simulink model "fftanalyzeri"  (R2012b)
settings: Solver=ode3  SolverMode=SingleTasking  StartTime=0.0  StopTime=20000  RelTol=1e-3
undefined symbols (not defined in the file or in its folder): pfb_coeff_gen_calc
undefined symbols (not defined in the file): fft_bin_flags_, magphmeanmem_, threshmem_
libraries: xbsIndex_r4 x9073, casper_library_misc x119, casper_library_flow_control x51, casper_library_delays x22, xps_library x10
(part 1 of 74)
settings Model: Creator=tmadden  LastModifiedBy=tmadden

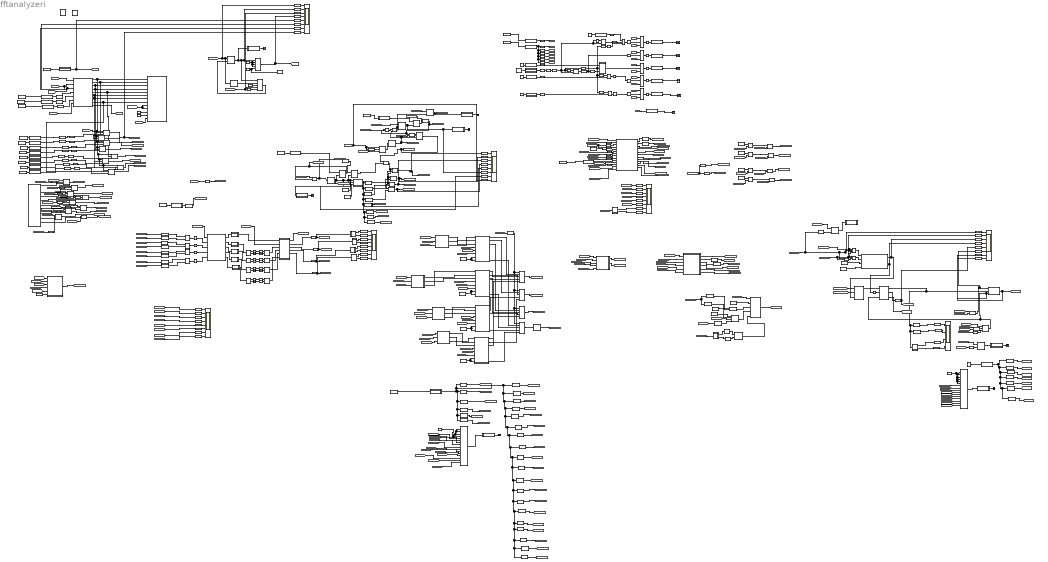
== system fftanalyzeri ==
  note: dumopFIFO is reallty read out fifos in proper wa to store fft data
  note: means fftcnt NOT done
  note: 32bits
  note: 32bits
  note: 32bits
  note: 32bits
  note: 7bits
  note: 0x55
  note: 16bits
  note: 16bits
  note: 16 bits
  note: 1bit
  note: 8 buts
  note: 0xaaaa
  note: 1st word fall thru
  note: 32 bit timestamp
  note: Now we put data backtogether
      | into 32bit buss
  note: This block extracts mag and phase
      | but truncates both numbers
      | to 16 bit.
  note: WE shrunk the mem to total of 32 bits
      | so we dont use all the bits in
      | header info.
      | all coef data go thru, but gets
      | truncated later...
      | we shoudl truncate here
      | to save resources...
  note: We truncate to 16bit data.
      | power is unsigned, all fraction bits
      | phase is signed w/ 13 frac bits
  note: This reg and bits are for
      | python user interface control
  note: if dropall evetns is 1 then save event and delete event will cause
      | a event to be deleted.
      | if drop all evetns is 0 then save event saves and delete events
      | deletes
  note: Because of bug in the fifos
      | we need extra delay on dvld.
      | we should out then in all
      | the underlying f16 chan fifos.
      | This is simpler for now...
  note: 1024 long
      | 32 bit wide
  note: 2 bits, sel 0,1,2,3 fifo
  note: Alolow fake ADC data to come into the system
  note: Counts number of FFTs forever
  note: if we want neg freq, that is freq below the rf carrier
      | we piuck eith coef 128-255 or 384 to 511
  note: ecause we cant read in whole fft we sel neg or pos freq
      | therefore we have a mux to give us coef 0-127 OR 256-383
  note: when startFFTs go high, cnt goes to state 0
      | when startFFt go low, cnt will goto state 1 because
      | of delayed 1 in delay19. counter gets to 2
      | and waits for lutsync, then goto 3.
      | it staty in 3 until we startFFTs again.
      | to shut ffts, set startFFTs high forever.
  note: Or a simulation input w/ HW input. the LIT is wierd in sumulation...
  note: go high to turn ffts mem storage off.
      | Go low to sync fft sunc to lut for phse reference
      | start fft saving
  note: states
      | 0	wait for fftstmem to go low, no fft sync
      | 1 waut for fftmemwe 0->1, no fft sunc
      | 2 wait for lut sync, no fft sunc
      | 3 fft sunc on, stay in this state forever
      |
      | fftstmem, forces fsm to state 0
  note: syscunc=1
      | startdac=0
      | startdac=1
      | syscunc=0
  note: if run_ffts is high, then the ffts run. else no ffts run.
  note: Read out FIFO state machine. Sauy we have 128 bins from fft. We read in groups of 4, w/ 4 outputs, so each fifo gets 32 bins
      | in each. So we will read out 32 numbers from each fifo. Counter counts from 0 to 127. LSBs pick which fifo.
      | There is a pipe line here. 1st we trigger FFT, which writes to FIFOS. Also we truggerm, assuming 1 fft pipeline delay
      | radoung out fifos. We have to read and write fifos same number of times or else we get out of sync
  note: The above is Ran's design for  ROACH IF baord
      | serial data stream. For programming IF board
      | clocks, gains, dividers.
  note: SWAT_LE
  note: LO_SLE
  note: SER_DI
  note: SER_CLK
  note: SW_STB
  note: Added by Tim Madden
  note: not in RANS design- below. Tim added the clk sle register so we can program the clocks
  note: bit 7
  note: CLK_SLE
  note: If bin>512, we disable any write fifo bits.
      | high if IS VALID bin number
  note: address for multi-fifo- which fifo does thei bin go into.
  note: Hight if we have computed less then N ffts
  note: just started daq, reset fft cnt to 0
  note: increments fft counter
  note: pulse for 1st fft done after starting daq
  note: pulse for every fft
  note: When high, we can write fifos, and read fifos, and wr end mdmory
  note: We can compute N ffts and stop storong.
      | This counts ffts stored.
      | Counter is reset on runffts going high,.
      | it is incremented every time we compute a fft.
  note: Set of 1's and 0;s in lsb
      | 1 to write that fft coef to fifos.
      | 4 outputs for fft, so we ave 4 bits
      | to det. if we write coef to fifo
  note: Bin counter.
      | inc for ecah bin from 0 to 511, or
      | mult of 512-1 up to 4k.when count
      | to 511, we write EVERY fft.
      | if we count to 1023, we write every other fft,
      | as long as the mem in BinData is 0 uip there.
      | We assume it is.
  note: high for each coef to write to fifo
  note: This is a pulse of 1 clk, for every group of coeffs to write. one pulse per ffft. goes 1 , 1clk before 1st coef
  note: This tunrs on after fftcuncout and staus on. as long as runffts is high.
  note: This Must be multiple of 512-1, like 511,1023,2047, max is 32 bits...
      | It can then skip FFTS, as higher mem on BinData is set to 0.
      | In thys way the 512 coef from FFT get written every Nth time. This is good if we wish to slow sample rate, or read whol FFT
      | Set to 512*5 - 1 to safely read all FFT coef.
  note: run_ffts is low, then q is 0.
      | run_ffts is hi, then q is one after fftsuncout.
      | this allows fifl wr
      | We can only write fifos when run_ffts is high.
      | fftoutsync comes some time after run-ffts goes high, when fft is done
  note: This is bin counter. it resets to 0 after 511, so it goes 0,1,2,3...511,0,1,2
      | it resets on fftsunc out, which happens once on reset at start of collection
  note: fftsyncout comes once at start of collection.
      | 1 clk lengthn pulse
      | it is for resetting and starting data collection
  note: Line up w/ data.
      | t1, fftdata0
      | tt4, phase 0
  note: fftsyncout_____________--________
  note: t=0,0
      | t=1,0
      | t=2,1
      | t=258,0
  note: at t=0, rst=1
      | t=1, cnt=0
      | t=2 cnt=1
      | t=257,cnt=256,
      | t=258...cnt=256
  note: FFT tap0: fft bin   04,8,etc.
      | tap 1  1,5,9...
      | tap 2   2,6,10...
      | tap3   3,7,11
  note: does mnothing.. set to 0
  note: run script fft_simvals.m to get this var
  note: 1 to let dac work
  note: make lut output the dram address instead if contents
  note: 1 to allow writing fft coef to fifos and output mem
  note: reset lut i think
  note: reset fft coef output mem addr to zero
  note: force fifo read to empty fifo of bad data
  note: loops back lut data into ffts, bypassing dac/adc etc
  note: set to 1 to make things run
  note: set whehc data gets saved to adc mem
  note: enable saving adc data to mem
  note: set adc wavemem addr to 0
  note: 1,0 will sync ffts w/ LUT and enable saving fft coef to ram
  note: Delay data, so we can save data befpre pulse was triggered
  note: Delay the data balid signal and data, so the pulse detector leads te actual data.
      | in this way we can detect pulse, shut off fifo, write header, then write the
      | 1st sample taht triggered pulse to memory
  note: Insert header data before pulse data.
      | We write just pulses to outptu memory.
      | So before pulse, we write magix number of 64k,
      | then write channel number,
      | then output pulse data.
  note: 32kx16bit
  note: 32K outptu fifo
      | uses ded. fifo
      | 32kwords * 4.5bytes/word=144kB
      | 16k length---> 72kB
  note: We read big fifo, and write to outram on this condition:
      | out ram is not full
      | we have NON empty fifo, that is, data is available from big fifo
      | We have enabled outmem writing w/ fftMemWE=1
  note: 1 when mem is full.
  note: fftMemWE enables reading 32K fifo into outram.
      | if memdone is high, we will not read the 32k fifo.
      | We read the big filo by
      | 1. fftMemWE<=0
      | 2. stFFTMem<=1
      | 3. stFFTMem<=0
      | 4 fftMemWE<=1
      | The fifo will be read, as long as there is data in it, until the outmem fills
      | or we set fftMemWE to 0.
      | When MemDone is 1, then we set fftMemWE to 0
      | We then copy memory w./ python over the network to linux.
      | Then we got to steo 1.
  note: 32k x 16bit
  note: Reset output mem addr to 0.
  note: wrout
  note: empty
  note: Output mempry that stores headers/pulse data.
      | Events to be written back to linux box.
  " System Generator" : xbsIndex_r4/ System Generator  Tag=genX  xilinxfamily=virtex5  part=xc5vsx95t  speed=-1  package=ff1136  synthesis_tool=XST  clock_wrapper=Clock Enables  directory=./fftanalyzeri/sysgen  proj_type=Project Navigator  Synth_file=XST Defaults  Impl_file=ISE Defaults  testbench=off  simulink_period=1  sysclk_period=7.8125  dcm_input_clock_period=100  incr_netlist=off  trim_vbits=Everywhere in SubSystem  dbl_ovrd=According to Block Masks  core_generation=According to Block Masks  run_coregen=off  deprecated_control=off  eval_field=0  block_type=sysgen
  Assert{,1..3} (4 alike) : xbsIndex_r4/Assert  assert_type=on  type_source=Explicitly  gui_display_data_type=Boolean  arith_type=Boolean  n_bits=16  bin_pt=14  preci_type=Single  exp_width=8  frac_width=24  assert_rate=on  rate_source=Explicitly  period=1  output_port=on  block_type=assert
  BinCounter : xbsIndex_r4/Counter  cnt_type=Free Running  cnt_to=Inf  operation=Up  start_count=0  cnt_by_val=1  arith_type=Unsigned  n_bits=32  bin_pt=0  load_pin=off  rst=on  en=off  explicit_period=on  period=1  dbl_ovrd=off  use_behavioral_HDL=off  implementation=Fabric  block_type=counter
  BinData : Subsystem  Tag=xps:bram  AncestorBlock=xps_library/Shared BRAM  mask{arith_type=Unsigned, addr_width=10, data_width=32, reg_prim_output=off, reg_core_output=off, optimization=Minimum_Area, data_bin_pt=0, init_vals=fft_bin_flags_, sample_rate=1}
      mask prompts: arith_type "Output Data Type"; addr_width "Address width"; data_width "Data Width"; reg_prim_output "Register Primitive Output"; reg_core_output "Register Core Output"; data_bin_pt "Data Binary Point"; init_vals "Initial values (simulation only)"; sample_rate "Sample rate"
      mask init:
      | shared_bram_mask;
      mask TypeOptions arith_type: Unsigned | Signed  (2's comp)
      mask TypeOptions data_width: 8 | 16 | 32 | 64 | 128
      mask TypeOptions optimization: Minimum_Area | Low_Power
  Concat : xbsIndex_r4/Concat  num_inputs=16  dbl_ovrd=off  block_type=concat
  Concat1 : xbsIndex_r4/Concat  num_inputs=4  dbl_ovrd=off  block_type=concat
  Concat2 : xbsIndex_r4/Concat  num_inputs=2  dbl_ovrd=off  block_type=concat
  Concat3 : xbsIndex_r4/Concat  num_inputs=16  dbl_ovrd=off  block_type=concat
  Concat4 : xbsIndex_r4/Concat  num_inputs=2  dbl_ovrd=off  block_type=concat
  Constant : xbsIndex_r4/Constant  const=0  gui_display_data_type=Boolean  arith_type=Boolean  n_bits=16  bin_pt=14  preci_type=Single  exp_width=8  frac_width=24  explicit_period=on  period=1  equ=P=C  opselect=C  inp2=PCIN>>17  opr=+  inp1=P  carry=CIN  dbl_ovrd=off  block_type=constant
  Constant1 : xbsIndex_r4/Constant  const=0  gui_display_data_type=Fixed-point  arith_type=Unsigned  n_bits=8  bin_pt=0  preci_type=Single  exp_width=8  frac_width=24  explicit_period=on  period=1  equ=P=C  opselect=C  inp2=PCIN>>17  opr=+  inp1=P  carry=CIN  dbl_ovrd=off  block_type=constant
  Constant10 : xbsIndex_r4/Constant  const=0  gui_display_data_type=Boolean  arith_type=Boolean  n_bits=4  bin_pt=0  preci_type=Single  exp_width=8  frac_width=24  explicit_period=on  period=1  equ=P=C  opselect=C  inp2=PCIN>>17  opr=+  inp1=P  carry=CIN  dbl_ovrd=off  block_type=constant
      settings: block_version=11.4
  Constant11 : Constant
  Constant12 : Constant  Value=2^31 + 2^29 + 2^15+2^4 + 2^0
  Constant14 : Constant
  Constant15 : Constant
  Constant2 : xbsIndex_r4/Constant  const=0  gui_display_data_type=Boolean  arith_type=Boolean  n_bits=4  bin_pt=0  preci_type=Single  exp_width=8  frac_width=24  explicit_period=on  period=1  equ=P=C  opselect=C  inp2=PCIN>>17  opr=+  inp1=P  carry=CIN  dbl_ovrd=off  block_type=constant
      settings: block_version=11.4
  Constant20 : xbsIndex_r4/Constant  const=0  gui_display_data_type=Boolean  arith_type=Boolean  n_bits=8  bin_pt=0  preci_type=Single  exp_width=8  frac_width=24  explicit_period=on  period=1  equ=P=C  opselect=C  inp2=PCIN>>17  opr=+  inp1=P  carry=CIN  dbl_ovrd=off  block_type=constant
  Constant24 : xbsIndex_r4/Constant  const=0  gui_display_data_type=Fixed-point  arith_type=Boolean  n_bits=4  bin_pt=0  preci_type=Single  exp_width=8  frac_width=24  explicit_period=on  period=1  equ=P=C  opselect=C  inp2=PCIN>>17  opr=+  inp1=P  carry=CIN  dbl_ovrd=off  block_type=constant
      settings: block_version=11.4
  Constant25 : xbsIndex_r4/Constant  const=1  gui_display_data_type=Boolean  arith_type=Boolean  n_bits=4  bin_pt=0  preci_type=Single  exp_width=8  frac_width=24  explicit_period=on  period=1  equ=P=C  opselect=C  inp2=PCIN>>17  opr=+  inp1=P  carry=CIN  dbl_ovrd=off  block_type=constant
      settings: block_version=11.4
  Constant26 : xbsIndex_r4/Constant  const=1  gui_display_data_type=Boolean  arith_type=Boolean  n_bits=4  bin_pt=0  preci_type=Single  exp_width=8  frac_width=24  explicit_period=on  period=1  equ=P=C  opselect=C  inp2=PCIN>>17  opr=+  inp1=P  carry=CIN  dbl_ovrd=off  block_type=constant
      settings: block_version=11.4
  Constant3 : Constant  Value=0
  Constant6 : xbsIndex_r4/Constant  const=0  gui_display_data_type=Fixed-point  arith_type=Boolean  n_bits=4  bin_pt=0  preci_type=Single  exp_width=8  frac_width=24  explicit_period=on  period=1  equ=P=C  opselect=C  inp2=PCIN>>17  opr=+  inp1=P  carry=CIN  dbl_ovrd=off  block_type=constant
      settings: block_version=11.4
  Constant7 : xbsIndex_r4/Constant  const=0  gui_display_data_type=Fixed-point  arith_type=Boolean  n_bits=4  bin_pt=0  preci_type=Single  exp_width=8  frac_width=24  explicit_period=on  period=1  equ=P=C  opselect=C  inp2=PCIN>>17  opr=+  inp1=P  carry=CIN  dbl_ovrd=off  block_type=constant
      settings: block_version=11.4
  Constant8 : xbsIndex_r4/Constant  const=0  gui_display_data_type=Fixed-point  arith_type=Unsigned  n_bits=4  bin_pt=0  preci_type=Single  exp_width=8  frac_width=24  explicit_period=on  period=1  equ=P=C  opselect=C  inp2=PCIN>>17  opr=+  inp1=P  carry=CIN  dbl_ovrd=off  block_type=constant
      settings: block_version=11.4
  Convert{4,6..12} (8 alike) : xbsIndex_r4/Convert  gui_display_data_type=Fixed-point  arith_type="Signed  (2's comp)"  n_bits=18  bin_pt=17  float_type=Single  exp_bits=8  fraction_bits=24  quantization="Round  (unbiased: +/- Inf)"  overflow=Wrap  en=off  latency=0  dbl_ovrd=off  pipeline=off  block_type=convert
      settings: xl_area=[0 0 0 0 0 0 0]  block_version=10.1.3
  Convert5 : xbsIndex_r4/Convert  gui_display_data_type=Fixed-point  arith_type=Unsigned  n_bits=33  bin_pt=0  float_type=Single  exp_bits=8  fraction_bits=24  quantization=Truncate  overflow=Wrap  en=off  latency=0  dbl_ovrd=off  pipeline=off  block_type=convert
      settings: block_version=11.4
  Counter2 : xbsIndex_r4/Counter  cnt_type=Free Running  cnt_to=2048  operation=Up  start_count=0  cnt_by_val=1  arith_type=Unsigned  n_bits=8  bin_pt=0  load_pin=off  rst=on  en=on  explicit_period=on  period=1  dbl_ovrd=off  use_behavioral_HDL=off  implementation=Fabric  use_rpm=off  block_type=counter
  Counter4 : xbsIndex_r4/Counter  cnt_type=Free Running  cnt_to=Inf  operation=Up  start_count=0  cnt_by_val=1  arith_type=Unsigned  n_bits=8  bin_pt=0  load_pin=off  rst=on  en=on  explicit_period=on  period=1  dbl_ovrd=off  use_behavioral_HDL=off  implementation=Fabric  block_type=counter
      settings: block_version=11.4
  DRAM_LUT : Subsystem
  DSbit0 : xbsIndex_r4/Slice  nbits=1  boolean_output=on  mode=Lower Bit Location + Width  bit1=0  base1=MSB of Input  bit0=0  base0=LSB of Input  dbl_ovrd=off  block_type=slice
  DSbit1 : xbsIndex_r4/Slice  nbits=1  boolean_output=on  mode=Lower Bit Location + Width  bit1=0  base1=MSB of Input  bit0=1  base0=LSB of Input  dbl_ovrd=off  block_type=slice
  DSbit2 : xbsIndex_r4/Slice  nbits=1  boolean_output=on  mode=Lower Bit Location + Width  bit1=0  base1=MSB of Input  bit0=2  base0=LSB of Input  dbl_ovrd=off  block_type=slice
  DSbit3 : xbsIndex_r4/Slice  nbits=1  boolean_output=on  mode=Lower Bit Location + Width  bit1=0  base1=MSB of Input  bit0=3  base0=LSB of Input  dbl_ovrd=off  block_type=slice
  DSbit4 : xbsIndex_r4/Slice  nbits=1  boolean_output=on  mode=Lower Bit Location + Width  bit1=0  base1=MSB of Input  bit0=4  base0=LSB of Input  dbl_ovrd=off  block_type=slice
  DSbit5 : xbsIndex_r4/Slice  nbits=1  boolean_output=on  mode=Lower Bit Location + Width  bit1=0  base1=MSB of Input  bit0=5  base0=LSB of Input  dbl_ovrd=off  block_type=slice
  DSbit6 : xbsIndex_r4/Slice  nbits=1  boolean_output=on  mode=Lower Bit Location + Width  bit1=0  base1=MSB of Input  bit0=6  base0=LSB of Input  dbl_ovrd=off  block_type=slice
  Delay{,2,9..16,18,20,29..32,34} (17 alike) : xbsIndex_r4/Delay  rst=off  infoeditControl=Selection of Reset will increase slice count due to use of real FFs and instead of SRLs  en=off  latency=1  dbl_ovrd=off  reg_retiming=off  block_type=delay
      Delay10 settings: xl_area=[18 36 0 0 0 0 0]
      Delay11 settings: xl_area=[18 36 0 0 0 0 0]
      Delay12 settings: xl_area=[18 36 0 0 0 0 0]
      Delay9 settings: xl_area=[18 36 0 0 0 0 0]
  Delay{1,3..8,17,19,21} (10 alike) : xbsIndex_r4/Delay  rst=off  infoeditControl=Selection of Reset will increase slice count due to use of real FFs and instead of SRLs  en=off  latency=2  dbl_ovrd=off  reg_retiming=off  block_type=delay
  Delay{23..24,27..28} (4 alike) : xbsIndex_r4/Delay  rst=off  infoeditControl=Selection of Reset will increase slice count due to use of real FFs and instead of SRLs  en=off  latency=64  dbl_ovrd=off  reg_retiming=off  block_type=delay
      settings: block_version=11.4
  EventLength : xbsIndex_r4/Constant  const=34  gui_display_data_type=Fixed-point  arith_type=Unsigned  n_bits=8  bin_pt=0  preci_type=Single  exp_width=8  frac_width=24  explicit_period=on  period=1  equ=P=C  opselect=C  inp2=PCIN>>17  opr=+  inp1=P  carry=CIN  dbl_ovrd=off  block_type=constant
  EventSaveFSM : xbsIndex_r4/MCode  mfname=eventsaveFSM  explicit_period=off  period=1  inputsTable={'boundInpExpr'=>['','','',''],'inputs'=>['save_event','delete_event','event_length','rst']}  outputsTable={'outputs'=>['eventfifo_rd','outfifo_wr'],'suppressOut'=>['off','off']}  dbl_ovrd=off  enable_stdout=off  enable_debug=off  suppress_output=on  defparams={}  hide_port_list={}  block_type=mcode
  EvtCnt : xbsIndex_r4/Counter  cnt_type=Free Running  cnt_to=Inf  operation=Up  start_count=0  cnt_by_val=1  arith_type=Unsigned  n_bits=32  bin_pt=0  load_pin=off  rst=on  en=on  explicit_period=on  period=1  dbl_ovrd=off  use_behavioral_HDL=off  implementation=Fabric  block_type=counter
  FIFO64_ : Subsystem
  FIFO64_1 : Subsystem
  FIFO64_2 : Subsystem
  FIFO64_3 : Subsystem
  From Workspace : FromWorkspace  VariableName=controlReg  OutDataTypeStr=double  SampleTime=1  Interpolate=off  OutputAfterFinalValue=Holding final value
  From Workspace1 : FromWorkspace  VariableName=if_switch  SampleTime=1  Interpolate=off  OutputAfterFinalValue=Holding final value
  From Workspace10 : FromWorkspace  VariableName=LUTsize  SampleTime=1  Interpolate=off  OutputAfterFinalValue=Holding final value
  From Workspace11 : FromWorkspace  VariableName=lut_i0  SampleTime=1  Interpolate=off  OutputAfterFinalValue=Holding final value
  From Workspace12 : FromWorkspace  VariableName=lut_i1  SampleTime=1  Interpolate=off  OutputAfterFinalValue=Holding final value
  From Workspace13 : FromWorkspace  VariableName=lut_i2  SampleTime=1  Interpolate=off  OutputAfterFinalValue=Holding final value
  From Workspace14 : FromWorkspace  VariableName=lut_i3  SampleTime=1  Interpolate=off  OutputAfterFinalValue=Holding final value
  From Workspace15 : FromWorkspace  VariableName=lut_q0  SampleTime=1  Interpolate=off  OutputAfterFinalValue=Holding final value
  From Workspace16 : FromWorkspace  VariableName=lut_q1  SampleTime=1  Interpolate=off  OutputAfterFinalValue=Holding final value
  From Workspace17 : FromWorkspace  VariableName=lut_q2  SampleTime=1  Interpolate=off  OutputAfterFinalValue=Holding final value
  From Workspace18 : FromWorkspace  VariableName=lut_q3  SampleTime=1  Interpolate=off  OutputAfterFinalValue=Holding final value
  From Workspace2 : FromWorkspace  VariableName=regs  SampleTime=1  Interpolate=off  OutputAfterFinalValue=Holding final value
  From Workspace3 : FromWorkspace  VariableName=lastChanToRead  SampleTime=1  Interpolate=off  OutputAfterFinalValue=Holding final value
  From Workspace4 : FromWorkspace  VariableName=numffts  SampleTime=1  Interpolate=off  OutputAfterFinalValue=Holding final value
  From Workspace5 : FromWorkspace  VariableName=fftsynctime  SampleTime=1  Interpolate=off  OutputAfterFinalValue=Holding final value
  From Workspace6 : FromWorkspace  VariableName=fftshift  SampleTime=1  Interpolate=off  OutputAfterFinalValue=Holding final value
  From Workspace7 : FromWorkspace  VariableName=resetDRAM  SampleTime=1  Interpolate=off  OutputAfterFinalValue=Holding final value
  From Workspace8 : FromWorkspace  VariableName=RWen  SampleTime=1  Interpolate=off  OutputAfterFinalValue=Holding final value
  From Workspace9 : FromWorkspace  VariableName=holdcounter  SampleTime=1  Interpolate=off  OutputAfterFinalValue=Holding final value
  Gateway Out{,1..51} (52 alike) : xbsIndex_r4/Gateway Out  inherit_from_input=off  hdl_port=on  timing_constraint=None  locs_specified=off  LOCs={}  UseAsDAC=off  DACChannel='1'  block_type=gatewayout
  Inverter{,1..6,8} (8 alike) : xbsIndex_r4/Inverter  en=off  latency=0  dbl_ovrd=off  block_type=inv
      Inverter1 settings: block_version=11.4
      Inverter2 settings: block_version=11.4
      Inverter3 settings: block_version=11.4
      Inverter4 settings: block_version=11.4
      Inverter5 settings: block_version=11.4
  LO_SLE : Subsystem  Tag=xps:sw_reg  AncestorBlock=xps_library/software register  mask{numios=1, io_dir=From Processor, io_delay=0, sample_period=1, name1=reg, bitwidth1=32, arith_type1=Unsigned, bin_pt1=0}
      mask prompts: numios "Num I/Os"; io_dir "I/O direction"; io_delay "I/O delay"; sample_period "Sample period"; name1 "Name"; bitwidth1 "Bitwidth"; arith_type1 "Type"; bin_pt1 "Binary pt"
      mask init:
      | swreg_init(gcb);
      mask Callback numios: t = timer('StartDelay', 0.1); t.TimerFcn = {@swreg_cb, gcb}; start(t);
      mask TypeOptions io_dir: To Processor | From Processor
      mask Callback io_dir:
      | a = get_param(gcb, 'MaskEnables');
      | if strcmp(get_param(gcb, 'io_dir'), 'To Processor'),
      | a(4) = {'off'};
      | else
      | a(4) = {'on'};
      | end
      | set_param(gcb, 'MaskEnables', a);
      mask TypeOptions arith_type1: Unsigned | Signed  (2's comp) | Boolean
      mask Callback arith_type1:
      | a = get_param(gcb, 'MaskEnables');
      | if strcmp(get_param(gcb, 'arith_type1'), 'Boolean'),
      | set_param(gcb, 'bitwidth1', '1');
      | set_param(gcb, 'bin_pt1', '0');
      | a(6) = {'off'};
      | a(8) = {'off'};
      | else
      | a(6) = {'on'};
      | a(8) = {'on'};
      | end
      | set_param(gcb, 'MaskEnables', a);
  LUTsize : Subsystem  Tag=xps:sw_reg  AncestorBlock=xps_library/software register  mask{numios=1, io_dir=From Processor, io_delay=0, sample_period=1, name1=reg, bitwidth1=32, arith_type1=Unsigned, bin_pt1=0}
      mask prompts: numios "Num I/Os"; io_dir "I/O direction"; io_delay "I/O delay"; sample_period "Sample period"; name1 "Name"; bitwidth1 "Bitwidth"; arith_type1 "Type"; bin_pt1 "Binary pt"
      mask init:
      | swreg_init(gcb);
      mask Callback numios: t = timer('StartDelay', 0.1); t.TimerFcn = {@swreg_cb, gcb}; start(t);
      mask TypeOptions io_dir: To Processor | From Processor
      mask Callback io_dir:
      | a = get_param(gcb, 'MaskEnables');
      | if strcmp(get_param(gcb, 'io_dir'), 'To Processor'),
      | a(4) = {'off'};
      | else
      | a(4) = {'on'};
      | end
      | set_param(gcb, 'MaskEnables', a);
      mask TypeOptions arith_type1: Unsigned | Signed  (2's comp) | Boolean
      mask Callback arith_type1:
      | a = get_param(gcb, 'MaskEnables');
      | if strcmp(get_param(gcb, 'arith_type1'), 'Boolean'),
      | set_param(gcb, 'bitwidth1', '1');
      | set_param(gcb, 'bin_pt1', '0');
      | a(6) = {'off'};
      | a(8) = {'off'};
      | else
      | a(6) = {'on'};
      | a(8) = {'on'};
      | end
      | set_param(gcb, 'MaskEnables', a);
  Logical : xbsIndex_r4/Logical  logical_function=AND  inputs=3  en=off  latency=0  precision=Full  arith_type=Unsigned  n_bits=16  bin_pt=0  align_bp=on  dbl_ovrd=off  block_type=logical
  Logical{1..3,14..17} (7 alike) : xbsIndex_r4/Logical  logical_function=OR  inputs=2  en=off  latency=0  precision=Full  arith_type=Unsigned  n_bits=16  bin_pt=0  align_bp=on  dbl_ovrd=off  block_type=logical
  Logical{4..8,10..13} (9 alike) : xbsIndex_r4/Logical  logical_function=AND  inputs=2  en=off  latency=0  precision=Full  arith_type=Unsigned  n_bits=16  bin_pt=0  align_bp=on  dbl_ovrd=off  block_type=logical
      Logical7 settings: block_version=11.4
      Logical8 settings: block_version=11.4
  Logical9 : xbsIndex_r4/Logical  logical_function=AND  inputs=3  en=off  latency=0  precision=Full  arith_type=Unsigned  n_bits=16  bin_pt=0  align_bp=on  dbl_ovrd=off  block_type=logical
      settings: block_version=11.4
  MCode1 : xbsIndex_r4/MCode  mfname=fifoFSMPh  explicit_period=on  period=1  inputsTable={'boundInpExpr'=>['','','','','','','','','','','','',''],'inputs'=>['dumpFifo','fifo_empty','half_full','quart_full','almost_full','rst','proc_busy','is_pulse','data_valid','last_channel','wr_raw_data','ram_pulse_state','is_calc_mean']}  outputsTable={'outputs'=>['fifo_rden','wr_coef_big_fifo','write_data_sel','cur_chanout','fifo_overrun_cnt_out','stateout','clear_pulse','datapath_enable','save_event','delete_event','save_pulse_state','calc_mean','store_mean'],'suppressOut'=>['off','off','off','off','off','off','off','off','off','off','off','off','off']}  dbl_ovrd=off  enable_stdout=off  enable_debug=off  suppress_output=on  defparams={}  hide_port_list={}  block_type=mcode
  MemRecordPolar : Subsystem
  Mux{,1..20} (21 alike) : xbsIndex_r4/Mux  inputs=2  en=off  latency=1  precision=Full  arith_type=Unsigned  n_bits=16  bin_pt=14  quantization=Truncate  overflow=Wrap  dbl_ovrd=off  block_type=mux
      Mux2 settings: block_version=11.4
      Mux3 settings: block_version=11.4
      Mux4 settings: block_version=11.4
      Mux5 settings: block_version=11.4
      Mux6 settings: block_version=11.4
  Mux21 : xbsIndex_r4/Mux  inputs=4  en=off  latency=0  precision=Full  arith_type=Unsigned  n_bits=16  bin_pt=14  quantization=Truncate  overflow=Wrap  dbl_ovrd=off  block_type=mux
  Mux22 : xbsIndex_r4/Mux  inputs=2  en=off  latency=0  precision=Full  arith_type=Unsigned  n_bits=16  bin_pt=14  quantization=Truncate  overflow=Wrap  dbl_ovrd=off  block_type=mux
  Mux23 : xbsIndex_r4/Mux  inputs=2  en=off  latency=0  precision=Full  arith_type=Unsigned  n_bits=16  bin_pt=14  quantization=Truncate  overflow=Wrap  dbl_ovrd=off  block_type=mux
  OutFIFO : xbsIndex_r4/FIFO  mem_type=Built-in FIFO  performance_options=First_Word_Fall_Through  infoedit1=Available only for V4, V5, V6, V7, K7, A7 and Zynq devices.  embedded_registers=off  depth=32K  percent_nbits=1  rst=off  en=off  use_dcount=off  use_percent_full_port=off  use_almost_empty=off  almost_empty_thresh=2  use_almost_full=off  almost_full_thresh=14  dbl_ovrd=off  explicit_period=off  block_type=fifo
  PhaseCorrect1 : Subsystem
  Pulse Generator2 : DiscretePulseGenerator  Period=11000  PulseWidth=10000  PhaseDelay=100
  PulseDetector : Subsystem
  RWen : Subsystem  Tag=xps:sw_reg  AncestorBlock=xps_library/software register  mask{numios=1, io_dir=From Processor, io_delay=0, sample_period=1, name1=reg, bitwidth1=32, arith_type1=Unsigned, bin_pt1=0}
      mask prompts: numios "Num I/Os"; io_dir "I/O direction"; io_delay "I/O delay"; sample_period "Sample period"; name1 "Name"; bitwidth1 "Bitwidth"; arith_type1 "Type"; bin_pt1 "Binary pt"
      mask init:
      | swreg_init(gcb);
      mask Callback numios: t = timer('StartDelay', 0.1); t.TimerFcn = {@swreg_cb, gcb}; start(t);
      mask TypeOptions io_dir: To Processor | From Processor
      mask Callback io_dir:
      | a = get_param(gcb, 'MaskEnables');
      | if strcmp(get_param(gcb, 'io_dir'), 'To Processor'),
      | a(4) = {'off'};
      | else
      | a(4) = {'on'};
      | end
      | set_param(gcb, 'MaskEnables', a);
      mask TypeOptions arith_type1: Unsigned | Signed  (2's comp) | Boolean
      mask Callback arith_type1:
      | a = get_param(gcb, 'MaskEnables');
      | if strcmp(get_param(gcb, 'arith_type1'), 'Boolean'),
      | set_param(gcb, 'bitwidth1', '1');
      | set_param(gcb, 'bin_pt1', '0');
      | a(6) = {'off'};
      | a(8) = {'off'};
      | else
      | a(6) = {'on'};
      | a(8) = {'on'};
      | end
      | set_param(gcb, 'MaskEnables', a);
  RectToPolar : Subsystem
  RectToPolar1 : Subsystem
  RectToPolar2 : Subsystem
  RectToPolar3 : Subsystem
  Register : xbsIndex_r4/Register  init=0  rst=on  en=on  dbl_ovrd=off  block_type=register
  Reinterpret{1..8} (8 alike) : xbsIndex_r4/Reinterpret  force_arith_type=off  arith_type="Signed  (2's comp)"  force_bin_pt=on  bin_pt=0  block_type=reinterpret
      settings: infoedit="Changes signal type without altering the binary representation.   You can changed the signal between signed and unsigned, and relocate the binary point.<br><br>Hardware notes: In hardware this block costs nothing.<br><br>Example:  Suppose the input is 6 bits wide, signed, with 2 fractional bits, and the output is forced to unsigned with 0 fractional bits.  Then an input of -2.0 (1110.00 in binary 2's complement) becomes an output of 56 (111000 in binary)."
  Relational{,1..2,5..6} (5 alike) : xbsIndex_r4/Relational  mode=a=b  en=off  latency=0  dbl_ovrd=off  block_type=relational
  Relational3 : xbsIndex_r4/Relational  mode=a!=b  en=off  latency=1  dbl_ovrd=off  block_type=relational
  Relational4 : xbsIndex_r4/Relational  mode=a>b  en=off  latency=0  dbl_ovrd=off  block_type=relational
  SER_DI : Subsystem  Tag=xps:sw_reg  AncestorBlock=xps_library/software register  mask{numios=1, io_dir=From Processor, io_delay=0, sample_period=1, name1=reg, bitwidth1=32, arith_type1=Unsigned, bin_pt1=0}
      mask prompts: numios "Num I/Os"; io_dir "I/O direction"; io_delay "I/O delay"; sample_period "Sample period"; name1 "Name"; bitwidth1 "Bitwidth"; arith_type1 "Type"; bin_pt1 "Binary pt"
      mask init:
      | swreg_init(gcb);
      mask Callback numios: t = timer('StartDelay', 0.1); t.TimerFcn = {@swreg_cb, gcb}; start(t);
      mask TypeOptions io_dir: To Processor | From Processor
      mask Callback io_dir:
      | a = get_param(gcb, 'MaskEnables');
      | if strcmp(get_param(gcb, 'io_dir'), 'To Processor'),
      | a(4) = {'off'};
      | else
      | a(4) = {'on'};
      | end
      | set_param(gcb, 'MaskEnables', a);
      mask TypeOptions arith_type1: Unsigned | Signed  (2's comp) | Boolean
      mask Callback arith_type1:
      | a = get_param(gcb, 'MaskEnables');
      | if strcmp(get_param(gcb, 'arith_type1'), 'Boolean'),
      | set_param(gcb, 'bitwidth1', '1');
      | set_param(gcb, 'bin_pt1', '0');
      | a(6) = {'off'};
      | a(8) = {'off'};
      | else
      | a(6) = {'on'};
      | a(8) = {'on'};
      | end
      | set_param(gcb, 'MaskEnables', a);
  SWAT_LE : Subsystem  Tag=xps:sw_reg  AncestorBlock=xps_library/software register  mask{numios=1, io_dir=From Processor, io_delay=0, sample_period=1, name1=reg, bitwidth1=32, arith_type1=Unsigned, bin_pt1=0}
      mask prompts: numios "Num I/Os"; io_dir "I/O direction"; io_delay "I/O delay"; sample_period "Sample period"; name1 "Name"; bitwidth1 "Bitwidth"; arith_type1 "Type"; bin_pt1 "Binary pt"
      mask init:
      | swreg_init(gcb);
      mask Callback numios: t = timer('StartDelay', 0.1); t.TimerFcn = {@swreg_cb, gcb}; start(t);
      mask TypeOptions io_dir: To Processor | From Processor
      mask Callback io_dir:
      | a = get_param(gcb, 'MaskEnables');
      | if strcmp(get_param(gcb, 'io_dir'), 'To Processor'),
      | a(4) = {'off'};
      | else
      | a(4) = {'on'};
      | end
      | set_param(gcb, 'MaskEnables', a);
      mask TypeOptions arith_type1: Unsigned | Signed  (2's comp) | Boolean
      mask Callback arith_type1:
      | a = get_param(gcb, 'MaskEnables');
      | if strcmp(get_param(gcb, 'arith_type1'), 'Boolean'),
      | set_param(gcb, 'bitwidth1', '1');
      | set_param(gcb, 'bin_pt1', '0');
      | a(6) = {'off'};
      | a(8) = {'off'};
      | else
      | a(6) = {'on'};
      | a(8) = {'on'};
      | end
      | set_param(gcb, 'MaskEnables', a);
  SinglaEvtFIFO1 : xbsIndex_r4/FIFO  mem_type=Built-in FIFO  performance_options=Standard_FIFO  infoedit1=Available only for V4, V5, V6, V7, K7, A7 and Zynq devices.  embedded_registers=off  depth=512  percent_nbits=1  rst=off  en=off  use_dcount=off  use_percent_full_port=off  use_almost_empty=off  almost_empty_thresh=2  use_almost_full=off  almost_full_thresh=14  dbl_ovrd=off  explicit_period=off  block_type=fifo
  Slice1 : xbsIndex_r4/Slice  nbits=1  boolean_output=on  mode=Lower Bit Location + Width  bit1=0  base1=MSB of Input  bit0=4  base0=LSB of Input  dbl_ovrd=off  block_type=slice
  Slice10 : xbsIndex_r4/Slice  nbits=1  boolean_output=on  mode=Upper Bit Location + Width  bit1=0  base1=MSB of Input  bit0=0  base0=LSB of Input  dbl_ovrd=off  block_type=slice
  Slice11 : xbsIndex_r4/Slice  nbits=1  boolean_output=on  mode=Lower Bit Location + Width  bit1=0  base1=MSB of Input  bit0=3  base0=LSB of Input  dbl_ovrd=off  block_type=slice
  Slice{13..15,20..21,23..24,26} (8 alike) : xbsIndex_r4/Slice  nbits=1  boolean_output=on  mode=Lower Bit Location + Width  bit1=0  base1=MSB of Input  bit0=0  base0=LSB of Input  dbl_ovrd=off  block_type=slice
      Slice13 settings: infoedit="Extracts a given range of bits from each input sample and presents it at the output.  The output type is ordinarily unsigned with binary point at zero, but can be Boolean when the slice is one bit wide.<P><P>Hardware notes: In hardware this block costs nothing."  block_version=10.1.3
      Slice23 settings: infoedit="Extracts a given range of bits from each input sample and presents it at the output.  The output type is ordinarily unsigned with binary point at zero, but can be Boolean when the slice is one bit wide.<P><P>Hardware notes: In hardware this block costs nothing."  block_version=10.1.3
      Slice24 settings: infoedit="Extracts a given range of bits from each input sample and presents it at the output.  The output type is ordinarily unsigned with binary point at zero, but can be Boolean when the slice is one bit wide.<P><P>Hardware notes: In hardware this block costs nothing."  block_version=10.1.3
  Slice2 : xbsIndex_r4/Slice  nbits=1  boolean_output=off  mode=Lower Bit Location + Width  bit1=0  base1=MSB of Input  bit0=0  base0=LSB of Input  dbl_ovrd=off  block_type=slice
  Slice22 : xbsIndex_r4/Slice  nbits=1  boolean_output=on  mode=Lower Bit Location + Width  bit1=0  base1=MSB of Input  bit0=1  base0=LSB of Input  dbl_ovrd=off  block_type=slice
  Slice25 : xbsIndex_r4/Slice  nbits=1  boolean_output=off  mode=Lower Bit Location + Width  bit1=0  base1=MSB of Input  bit0=2  base0=LSB of Input  dbl_ovrd=off  block_type=slice
  Slice3 : xbsIndex_r4/Slice  nbits=7  boolean_output=on  mode=Lower Bit Location + Width  bit1=0  base1=MSB of Input  bit0=0  base0=MSB of Input  dbl_ovrd=off  block_type=slice
      settings: block_version=10.1.3
  Slice4 : xbsIndex_r4/Slice  nbits=1  boolean_output=on  mode=Lower Bit Location + Width  bit1=0  base1=MSB of Input  bit0=5  base0=LSB of Input  dbl_ovrd=off  block_type=slice
  TSHi : xbsIndex_r4/Slice  nbits=16  boolean_output=off  mode=Lower Bit Location + Width  bit1=0  base1=MSB of Input  bit0=16  base0=LSB of Input  dbl_ovrd=off  block_type=slice
  TSHi1 : xbsIndex_r4/Slice  nbits=16  boolean_output=off  mode=Lower Bit Location + Width  bit1=0  base1=MSB of Input  bit0=16  base0=LSB of Input  dbl_ovrd=off  block_type=slice
  TSLow : xbsIndex_r4/Slice  nbits=16  boolean_output=off  mode=Lower Bit Location + Width  bit1=0  base1=MSB of Input  bit0=0  base0=LSB of Input  dbl_ovrd=off  block_type=slice
  TSLow1 : xbsIndex_r4/Slice  nbits=16  boolean_output=off  mode=Lower Bit Location + Width  bit1=0  base1=MSB of Input  bit0=0  base0=LSB of Input  dbl_ovrd=off  block_type=slice
  Terminator{,1..12} (13 alike) : Terminator
  XSG core config : xps_library/XSG core config  Tag=xps:xsg  hw_sys=ROACH:sx95t  clk_src=adc1_clk  ROACH_clk_src=adc1_clk  ROACH2_clk_src=adc0_clk  clk_rate=128  sample_period=1  synthesis_tool=XST
  adcWaveMem : Subsystem
  adc_mkid_4x : xps_library/ADCs/adc_mkid_4x  Tag=xps:adc_mkid_4x  adc_brd=1  adc_clk_rate=512
  bincount_out : Subsystem  Tag=xps:sw_reg  AncestorBlock=xps_library/software register  mask{numios=1, io_dir=To Processor, io_delay=0, sample_period=1, name1=reg, bitwidth1=32, arith_type1=Unsigned, bin_pt1=0}
      mask prompts: numios "Num I/Os"; io_dir "I/O direction"; io_delay "I/O delay"; sample_period "Sample period"; name1 "Name"; bitwidth1 "Bitwidth"; arith_type1 "Type"; bin_pt1 "Binary pt"
      mask init:
      | swreg_init(gcb);
      mask Callback numios: t = timer('StartDelay', 0.1); t.TimerFcn = {@swreg_cb, gcb}; start(t);
      mask TypeOptions io_dir: To Processor | From Processor
      mask Callback io_dir:
      | a = get_param(gcb, 'MaskEnables');
      | if strcmp(get_param(gcb, 'io_dir'), 'To Processor'),
      | a(4) = {'off'};
      | else
      | a(4) = {'on'};
      | end
      | set_param(gcb, 'MaskEnables', a);
      mask TypeOptions arith_type1: Unsigned | Signed  (2's comp) | Boolean
      mask Callback arith_type1:
      | a = get_param(gcb, 'MaskEnables');
      | if strcmp(get_param(gcb, 'arith_type1'), 'Boolean'),
      | set_param(gcb, 'bitwidth1', '1');
      | set_param(gcb, 'bin_pt1', '0');
      | a(6) = {'off'};
      | a(8) = {'off'};
      | else
      | a(6) = {'on'};
      | a(8) = {'on'};
      | end
      | set_param(gcb, 'MaskEnables', a);
  bit0 : xbsIndex_r4/Slice  nbits=1  boolean_output=on  mode=Lower Bit Location + Width  bit1=0  base1=MSB of Input  bit0=0  base0=LSB of Input  dbl_ovrd=off  block_type=slice
  bit1 : xbsIndex_r4/Slice  nbits=1  boolean_output=on  mode=Lower Bit Location + Width  bit1=0  base1=MSB of Input  bit0=1  base0=LSB of Input  dbl_ovrd=off  block_type=slice
  bit12 : xbsIndex_r4/Slice  nbits=1  boolean_output=on  mode=Lower Bit Location + Width  bit1=0  base1=MSB of Input  bit0=12  base0=LSB of Input  dbl_ovrd=off  block_type=slice
  bit13 : xbsIndex_r4/Slice  nbits=1  boolean_output=on  mode=Lower Bit Location + Width  bit1=0  base1=MSB of Input  bit0=13  base0=LSB of Input  dbl_ovrd=off  block_type=slice
  bit14 : xbsIndex_r4/Slice  nbits=1  boolean_output=on  mode=Lower Bit Location + Width  bit1=0  base1=MSB of Input  bit0=14  base0=LSB of Input  dbl_ovrd=off  block_type=slice
  bit15 : xbsIndex_r4/Slice  nbits=1  boolean_output=on  mode=Lower Bit Location + Width  bit1=0  base1=MSB of Input  bit0=15  base0=LSB of Input  dbl_ovrd=off  block_type=slice
  bit16 : xbsIndex_r4/Slice  nbits=1  boolean_output=on  mode=Lower Bit Location + Width  bit1=0  base1=MSB of Input  bit0=16  base0=LSB of Input  dbl_ovrd=off  block_type=slice
  bit17 : xbsIndex_r4/Slice  nbits=1  boolean_output=on  mode=Lower Bit Location + Width  bit1=0  base1=MSB of Input  bit0=17  base0=LSB of Input  dbl_ovrd=off  block_type=slice
  bit18 : xbsIndex_r4/Slice  nbits=1  boolean_output=on  mode=Lower Bit Location + Width  bit1=0  base1=MSB of Input  bit0=18  base0=LSB of Input  dbl_ovrd=off  block_type=slice
  bit19 : xbsIndex_r4/Slice  nbits=1  boolean_output=on  mode=Lower Bit Location + Width  bit1=0  base1=MSB of Input  bit0=19  base0=LSB of Input  dbl_ovrd=off  block_type=slice
  bit2 : xbsIndex_r4/Slice  nbits=1  boolean_output=on  mode=Lower Bit Location + Width  bit1=0  base1=MSB of Input  bit0=2  base0=LSB of Input  dbl_ovrd=off  block_type=slice
  bit20 : xbsIndex_r4/Slice  nbits=1  boolean_output=on  mode=Lower Bit Location + Width  bit1=0  base1=MSB of Input  bit0=20  base0=LSB of Input  dbl_ovrd=off  block_type=slice
  bit21 : xbsIndex_r4/Slice  nbits=1  boolean_output=on  mode=Lower Bit Location + Width  bit1=0  base1=MSB of Input  bit0=21  base0=LSB of Input  dbl_ovrd=off  block_type=slice
  bit22 : xbsIndex_r4/Slice  nbits=1  boolean_output=on  mode=Lower Bit Location + Width  bit1=0  base1=MSB of Input  bit0=22  base0=LSB of Input  dbl_ovrd=off  block_type=slice
  bit23 : xbsIndex_r4/Slice  nbits=1  boolean_output=on  mode=Lower Bit Location + Width  bit1=0  base1=MSB of Input  bit0=23  base0=LSB of Input  dbl_ovrd=off  block_type=slice
  bit24 : xbsIndex_r4/Slice  nbits=1  boolean_output=on  mode=Lower Bit Location + Width  bit1=0  base1=MSB of Input  bit0=24  base0=LSB of Input  dbl_ovrd=off  block_type=slice
  bit25 : xbsIndex_r4/Slice  nbits=1  boolean_output=on  mode=Lower Bit Location + Width  bit1=0  base1=MSB of Input  bit0=25  base0=LSB of Input  dbl_ovrd=off  block_type=slice
  bit26 : xbsIndex_r4/Slice  nbits=1  boolean_output=on  mode=Lower Bit Location + Width  bit1=0  base1=MSB of Input  bit0=26  base0=LSB of Input  dbl_ovrd=off  block_type=slice
  bit3 : xbsIndex_r4/Slice  nbits=1  boolean_output=on  mode=Lower Bit Location + Width  bit1=0  base1=MSB of Input  bit0=3  base0=LSB of Input  dbl_ovrd=off  block_type=slice
  bit4 : xbsIndex_r4/Slice  nbits=1  boolean_output=on  mode=Lower Bit Location + Width  bit1=0  base1=MSB of Input  bit0=4  base0=LSB of Input  dbl_ovrd=off  block_type=slice
  bit5 : xbsIndex_r4/Slice  nbits=1  boolean_output=on  mode=Lower Bit Location + Width  bit1=0  base1=MSB of Input  bit0=5  base0=LSB of Input  dbl_ovrd=off  block_type=slice
  bit6 : xbsIndex_r4/Slice  nbits=1  boolean_output=on  mode=Lower Bit Location + Width  bit1=0  base1=MSB of Input  bit0=6  base0=LSB of Input  dbl_ovrd=off  block_type=slice
  bit7 : xbsIndex_r4/Slice  nbits=1  boolean_output=on  mode=Lower Bit Location + Width  bit1=0  base1=MSB of Input  bit0=7  base0=LSB of Input  dbl_ovrd=off  block_type=slice
  bit8 : xbsIndex_r4/Slice  nbits=1  boolean_output=on  mode=Lower Bit Location + Width  bit1=0  base1=MSB of Input  bit0=8  base0=LSB of Input  dbl_ovrd=off  block_type=slice
  bit9__ : xbsIndex_r4/Slice  nbits=1  boolean_output=off  mode=Lower Bit Location + Width  bit1=0  base1=MSB of Input  bit0=9  base0=LSB of Input  dbl_ovrd=off  block_type=slice
  bits2_ : xbsIndex_r4/Constant  const=0  gui_display_data_type=Fixed-point  arith_type=Unsigned  n_bits=2  bin_pt=0  preci_type=Single  exp_width=8  frac_width=24  explicit_period=on  period=1  equ=P=C  opselect=C  inp2=PCIN>>17  opr=+  inp1=P  carry=CIN  dbl_ovrd=off  block_type=constant
  bits2_1 : xbsIndex_r4/Constant  const=1  gui_display_data_type=Fixed-point  arith_type=Unsigned  n_bits=2  bin_pt=0  preci_type=Single  exp_width=8  frac_width=24  explicit_period=on  period=1  equ=P=C  opselect=C  inp2=PCIN>>17  opr=+  inp1=P  carry=CIN  dbl_ovrd=off  block_type=constant
  bits2_2 : xbsIndex_r4/Constant  const=2  gui_display_data_type=Fixed-point  arith_type=Unsigned  n_bits=2  bin_pt=0  preci_type=Single  exp_width=8  frac_width=24  explicit_period=on  period=1  equ=P=C  opselect=C  inp2=PCIN>>17  opr=+  inp1=P  carry=CIN  dbl_ovrd=off  block_type=constant
  bits2_3 : xbsIndex_r4/Constant  const=3  gui_display_data_type=Fixed-point  arith_type=Unsigned  n_bits=2  bin_pt=0  preci_type=Single  exp_width=8  frac_width=24  explicit_period=on  period=1  equ=P=C  opselect=C  inp2=PCIN>>17  opr=+  inp1=P  carry=CIN  dbl_ovrd=off  block_type=constant
  bits76_ : xbsIndex_r4/Slice  nbits=2  boolean_output=off  mode=Lower Bit Location + Width  bit1=0  base1=MSB of Input  bit0=6  base0=LSB of Input  dbl_ovrd=off  block_type=slice
  bits_0_11_ : xbsIndex_r4/Slice  nbits=11  boolean_output=off  mode=Lower Bit Location + Width  bit1=0  base1=MSB of Input  bit0=0  base0=LSB of Input  dbl_ovrd=off  block_type=slice
  bool_{,1..2,4..8} (8 alike) : xbsIndex_r4/Assert  assert_type=on  type_source=Explicitly  gui_display_data_type=Boolean  arith_type=Boolean  n_bits=16  bin_pt=14  preci_type=Single  exp_width=8  frac_width=24  assert_rate=on  rate_source=Explicitly  period=1  output_port=on  block_type=assert
  bool_100 : xbsIndex_r4/Constant  const=0  gui_display_data_type=Boolean  arith_type=Boolean  n_bits=16  bin_pt=14  preci_type=Single  exp_width=8  frac_width=24  explicit_period=on  period=1  equ=P=C  opselect=C  inp2=PCIN>>17  opr=+  inp1=P  carry=CIN  dbl_ovrd=off  block_type=constant
  c2Polar16_2 : Subsystem
  c2TruncatePolar16_1 : Subsystem
  c2polar_ : Subsystem
  c2polar_1 : Subsystem
  c2polar_2 : Subsystem
  c2polar_3 : Subsystem
  c2polar_5 : Subsystem
  c_to_ri{,1..3} (4 alike) : casper_library_misc/c_to_ri  n_bits=12  bin_pt=11
      settings: AttributesFormatString=12_11 r/i
  coefWrEn_and_validbin : xbsIndex_r4/Logical  logical_function=AND  inputs=2  en=off  latency=0  precision=Full  arith_type=Unsigned  n_bits=16  bin_pt=0  align_bp=on  dbl_ovrd=off  block_type=logical
  coefbit0_ : xbsIndex_r4/Slice  nbits=1  boolean_output=on  mode=Lower Bit Location + Width  bit1=0  base1=MSB of Input  bit0=0  base0=LSB of Input  dbl_ovrd=off  block_type=slice
  coefbit1_ : xbsIndex_r4/Slice  nbits=1  boolean_output=on  mode=Lower Bit Location + Width  bit1=0  base1=MSB of Input  bit0=1  base0=LSB of Input  dbl_ovrd=off  block_type=slice
  coefbit2_ : xbsIndex_r4/Slice  nbits=1  boolean_output=on  mode=Lower Bit Location + Width  bit1=0  base1=MSB of Input  bit0=2  base0=LSB of Input  dbl_ovrd=off  block_type=slice
  coefbit3_ : xbsIndex_r4/Slice  nbits=1  boolean_output=on  mode=Lower Bit Location + Width  bit1=0  base1=MSB of Input  bit0=3  base0=LSB of Input  dbl_ovrd=off  block_type=slice
  controlReg : Subsystem  Tag=xps:sw_reg  AncestorBlock=xps_library/software register  mask{numios=1, io_dir=From Processor, io_delay=0, sample_period=1, name1=reg, bitwidth1=32, arith_type1=Unsigned, bin_pt1=0}
      mask prompts: numios "Num I/Os"; io_dir "I/O direction"; io_delay "I/O delay"; sample_period "Sample period"; name1 "Name"; bitwidth1 "Bitwidth"; arith_type1 "Type"; bin_pt1 "Binary pt"
      mask init:
      | swreg_init(gcb);
      mask Callback numios: t = timer('StartDelay', 0.1); t.TimerFcn = {@swreg_cb, gcb}; start(t);
      mask TypeOptions io_dir: To Processor | From Processor
      mask Callback io_dir:
      | a = get_param(gcb, 'MaskEnables');
      | if strcmp(get_param(gcb, 'io_dir'), 'To Processor'),
      | a(4) = {'off'};
      | else
      | a(4) = {'on'};
      | end
      | set_param(gcb, 'MaskEnables', a);
      mask TypeOptions arith_type1: Unsigned | Signed  (2's comp) | Boolean
      mask Callback arith_type1:
      | a = get_param(gcb, 'MaskEnables');
      | if strcmp(get_param(gcb, 'arith_type1'), 'Boolean'),
      | set_param(gcb, 'bitwidth1', '1');
      | set_param(gcb, 'bin_pt1', '0');
      | a(6) = {'off'};
      | a(8) = {'off'};
      | else
      | a(6) = {'on'};
      | a(8) = {'on'};
      | end
      | set_param(gcb, 'MaskEnables', a);
  count_2bit : xbsIndex_r4/Counter  cnt_type=Free Running  cnt_to=Inf  operation=Up  start_count=0  cnt_by_val=1  arith_type=Unsigned  n_bits=2  bin_pt=0  load_pin=off  rst=on  en=on  explicit_period=on  period=1  dbl_ovrd=off  use_behavioral_HDL=off  implementation=Fabric  block_type=counter
  dac_mkid_4x : xps_library/DACs/dac_mkid_4x  Tag=xps:dac_mkid_4x  dac_brd=0  dac_clk_rate=512  sample_period=1
  dacscope : Scope  NumInputPorts=8
      settings: YMin=-5~-5~-5~-5~-5~-5~-5~-5  YMax=5~5~5~5~5~5~5~5  SaveName=fsmdata11
  datamux : xbsIndex_r4/Mux  inputs=4  en=off  latency=0  precision=Full  arith_type=Unsigned  n_bits=16  bin_pt=14  quantization=Truncate  overflow=Wrap  dbl_ovrd=off  block_type=mux
  edgdet : casper_library_misc/edge_detect  edge=Rising  polarity=Active High  x_in=[0 0.08 0.08 0.16 0.16 0.24 0.24 0.32 0.32 0.4]  y_in="[-1 -1  1  1  1  1  1  1  1  1]"  x_out=[0.6 0.68 0.68 0.76 0.76 0.84 0.84 0.92 0.92 1]  y_out="[-1 -1  1  1 -1 -1 -1 -1 -1 -1]"
  emptymux : xbsIndex_r4/Mux  inputs=4  en=off  latency=0  precision=Full  arith_type=Unsigned  n_bits=16  bin_pt=14  quantization=Truncate  overflow=Wrap  dbl_ovrd=off  block_type=mux
  fft1 : Subsystem  AncestorBlock=casper_library_ffts/fft  mask(fft){n_streams=1, FFTSize=9, n_inputs=2, input_bit_width=18, bin_pt_in=-1, coeff_bit_width=18, async=off, unscramble=on, add_latency=1, mult_latency=2, bram_latency=2, conv_latency=1, quantization=Round  (unbiased: +/- Inf), overflow=Saturate, delays_bit_limit=8, coeffs_bit_limit=9, coeff_sharing=on, coeff_decimation=on, coeff_generation=on, cal_bits=1, n_bits_rotation=25, max_fanout=4, mult_spec=2, bitgrowth=off, max_bits=19, hardcode_shifts=off, shift_schedule=, dsp48_adders=off}
      mask prompts: n_streams "Number input streams"; FFTSize "Size of FFT: (2^? pts)"; n_inputs "Number of Simultaneous Inputs: (2^?)"; input_bit_width "Input bit width"; bin_pt_in "Input binary point"; coeff_bit_width "Coefficient Bit Width"; async "Asynchronous operation"; unscramble "Unscramble output (ie, put channels in canonical order)"; add_latency "Add Latency"; mult_latency "Mult Latency"; bram_latency "BRAM Latency"; conv_latency "Convert Latency"; quantization "Quantization Behavior"; overflow "Overflow Behavior"; delays_bit_limit "Number bits above which to store stage's delays in BRAM (2^? bits)"; coeffs_bit_limit "Number bits above which to store stage's coefficients in BRAM (2^? bits)"; coeff_sharing "BRAM sharing in coeff storage"; coeff_decimation "Store a fraction of coeff factors where useful"; coeff_generation "Generate coeffs with multipliers where useful"; cal_bits "Number calibration locations when generating coeffs (2^?)"; n_bits_rotation "Feedback rotation vector resolution"; max_fanout "Maximum fanout"; mult_spec "Multiplier impl. (0=core, 1=embedded, 2=behavioural) (left=1st stage, or just one value)"; bitgrowth "Bitgrowth instead of shifting"; max_bits "Max bits to grow to"; hardcode_shifts "Hardcode shift schedule"; shift_schedule "Shift schedule"; dsp48_adders "DSP48 adders in butterfly"
      mask help: A complex FFT.
      mask init:
      | fft_init(gcb, ...
      |     'n_streams', n_streams, ...
      |     'FFTSize', FFTSize, ...
      |     'n_inputs', n_inputs, ...
      |     'input_bit_width', input_bit_width, ...
      |     'coeff_bit_width', coeff_bit_width, ...
      |     'async', async, ...
      |     'unscramble', unscramble, ...
      |     'add_latency', add_latency, ...
      |     'mult_latency', mult_latency, ...
      |     'bram_latency', bram_latency, ...
      |     'conv_latency', conv_latency, ...
      |     'quantization', quantization, ...
      |     'overflow', overflow, ...
      |     'delays_bit_limit', delays_bit_limit, ...
      |     'coeffs_bit_limit', coeffs_bit_limit, ...
      |     'coeff_sharing', coeff_sharing, ...
      |     'coeff_decimation', coeff_decimation, ...
      |     'coeff_generation', coeff_generation, ...
      |     'cal_bits', cal_bits, ...
      |     'n_bits_rotation', n_bits_rotation, ...
      |     'max_fanout', max_fanout, ...   
      |     'mult_spec', mult_spec, ...
      |     'bitgrowth', bitgrowth, ...
      |     'hardcode_shifts', hardcode_shifts, ...
      |     'shift_schedule', shift_schedule, ...
      |     'dsp48_adders', dsp48_adders);
      settings: AttributesFormatString=|
      | 9 stages
      | (18,18)
      | Round  (unbiased: +/- Inf)
      | Saturate
      mask Help: eval('xlWeb(''http://casper.berkeley.edu/wiki/Fft'')')
      mask TypeOptions quantization: Truncate | Round  (unbiased: +/- Inf) | Round  (unbiased: Even Values)
      mask TypeOptions overflow: Wrap | Saturate | Error
      mask Callback hardcode_shifts:
      | hardcode_shifts = get_param(gcb, 'hardcode_shifts');
      | set_param_state(gcb, 'shift_schedule', hardcode_shifts);
      mask Callback dsp48_adders: fft_callback_dsp48_adders(gcb);
  fftcounter : xbsIndex_r4/Counter  cnt_type=Free Running  cnt_to=Inf  operation=Up  start_count=0  cnt_by_val=1  arith_type=Unsigned  n_bits=32  bin_pt=0  load_pin=off  rst=on  en=on  explicit_period=on  period=1  dbl_ovrd=off  use_behavioral_HDL=off  implementation=Fabric  block_type=counter
  fftcounter_out : Subsystem  Tag=xps:sw_reg  AncestorBlock=xps_library/software register  mask{numios=1, io_dir=To Processor, io_delay=0, sample_period=1, name1=reg, bitwidth1=32, arith_type1=Unsigned, bin_pt1=0}
      mask prompts: numios "Num I/Os"; io_dir "I/O direction"; io_delay "I/O delay"; sample_period "Sample period"; name1 "Name"; bitwidth1 "Bitwidth"; arith_type1 "Type"; bin_pt1 "Binary pt"
      mask init:
      | swreg_init(gcb);
      mask Callback numios: t = timer('StartDelay', 0.1); t.TimerFcn = {@swreg_cb, gcb}; start(t);
      mask TypeOptions io_dir: To Processor | From Processor
      mask Callback io_dir:
      | a = get_param(gcb, 'MaskEnables');
      | if strcmp(get_param(gcb, 'io_dir'), 'To Processor'),
      | a(4) = {'off'};
      | else
      | a(4) = {'on'};
      | end
      | set_param(gcb, 'MaskEnables', a);
      mask TypeOptions arith_type1: Unsigned | Signed  (2's comp) | Boolean
      mask Callback arith_type1:
      | a = get_param(gcb, 'MaskEnables');
      | if strcmp(get_param(gcb, 'arith_type1'), 'Boolean'),
      | set_param(gcb, 'bitwidth1', '1');
      | set_param(gcb, 'bin_pt1', '0');
      | a(6) = {'off'};
      | a(8) = {'off'};
      | else
      | a(6) = {'on'};
      | a(8) = {'on'};
      | end
      | set_param(gcb, 'MaskEnables', a);
  fftscope : Scope  NumInputPorts=8
      settings: YMin=-5~-5~-5~-5~-5~-5~-5~-5  YMax=5~5~5~5~5~5~5~5  SaveName=fsmdata3
  fftscope1 : Scope  NumInputPorts=8
      settings: YMin=-5~-5~-5~-5~-5~-5~-5~-5  YMax=5~5~5~5~5~5~5~5  SaveName=fsmdata9
  fftshift : Subsystem  Tag=xps:sw_reg  AncestorBlock=xps_library/software register  mask{numios=1, io_dir=From Processor, io_delay=0, sample_period=1, name1=reg, bitwidth1=32, arith_type1=Unsigned, bin_pt1=0}
      mask prompts: numios "Num I/Os"; io_dir "I/O direction"; io_delay "I/O delay"; sample_period "Sample period"; name1 "Name"; bitwidth1 "Bitwidth"; arith_type1 "Type"; bin_pt1 "Binary pt"
      mask init:
      | swreg_init(gcb);
      mask Callback numios: t = timer('StartDelay', 0.1); t.TimerFcn = {@swreg_cb, gcb}; start(t);
      mask TypeOptions io_dir: To Processor | From Processor
      mask Callback io_dir:
      | a = get_param(gcb, 'MaskEnables');
      | if strcmp(get_param(gcb, 'io_dir'), 'To Processor'),
      | a(4) = {'off'};
      | else
      | a(4) = {'on'};
      | end
      | set_param(gcb, 'MaskEnables', a);
      mask TypeOptions arith_type1: Unsigned | Signed  (2's comp) | Boolean
      mask Callback arith_type1:
      | a = get_param(gcb, 'MaskEnables');
      | if strcmp(get_param(gcb, 'arith_type1'), 'Boolean'),
      | set_param(gcb, 'bitwidth1', '1');
      | set_param(gcb, 'bin_pt1', '0');
      | a(6) = {'off'};
      | a(8) = {'off'};
      | else
      | a(6) = {'on'};
      | a(8) = {'on'};
      | end
      | set_param(gcb, 'MaskEnables', a);
  fftsynctime : Subsystem  Tag=xps:sw_reg  AncestorBlock=xps_library/software register  mask{numios=1, io_dir=From Processor, io_delay=0, sample_period=1, name1=reg, bitwidth1=32, arith_type1=Unsigned, bin_pt1=0}
      mask prompts: numios "Num I/Os"; io_dir "I/O direction"; io_delay "I/O delay"; sample_period "Sample period"; name1 "Name"; bitwidth1 "Bitwidth"; arith_type1 "Type"; bin_pt1 "Binary pt"
      mask init:
      | swreg_init(gcb);
      mask Callback numios: t = timer('StartDelay', 0.1); t.TimerFcn = {@swreg_cb, gcb}; start(t);
      mask TypeOptions io_dir: To Processor | From Processor
      mask Callback io_dir:
      | a = get_param(gcb, 'MaskEnables');
      | if strcmp(get_param(gcb, 'io_dir'), 'To Processor'),
      | a(4) = {'off'};
      | else
      | a(4) = {'on'};
      | end
      | set_param(gcb, 'MaskEnables', a);
      mask TypeOptions arith_type1: Unsigned | Signed  (2's comp) | Boolean
      mask Callback arith_type1:
      | a = get_param(gcb, 'MaskEnables');
      | if strcmp(get_param(gcb, 'arith_type1'), 'Boolean'),
      | set_param(gcb, 'bitwidth1', '1');
      | set_param(gcb, 'bin_pt1', '0');
      | a(6) = {'off'};
      | a(8) = {'off'};
      | else
      | a(6) = {'on'};
      | a(8) = {'on'};
      | end
      | set_param(gcb, 'MaskEnables', a);
  fifoOverFlowCnt : Subsystem  Tag=xps:sw_reg  AncestorBlock=xps_library/software register  mask{numios=1, io_dir=To Processor, io_delay=0, sample_period=1, name1=reg, bitwidth1=32, arith_type1=Unsigned, bin_pt1=0}
      mask prompts: numios "Num I/Os"; io_dir "I/O direction"; io_delay "I/O delay"; sample_period "Sample period"; name1 "Name"; bitwidth1 "Bitwidth"; arith_type1 "Type"; bin_pt1 "Binary pt"
      mask init:
      | swreg_init(gcb);
      mask Callback numios: t = timer('StartDelay', 0.1); t.TimerFcn = {@swreg_cb, gcb}; start(t);
      mask TypeOptions io_dir: To Processor | From Processor
      mask Callback io_dir:
      | a = get_param(gcb, 'MaskEnables');
      | if strcmp(get_param(gcb, 'io_dir'), 'To Processor'),
      | a(4) = {'off'};
      | else
      | a(4) = {'on'};
      | end
      | set_param(gcb, 'MaskEnables', a);
      mask TypeOptions arith_type1: Unsigned | Signed  (2's comp) | Boolean
      mask Callback arith_type1:
      | a = get_param(gcb, 'MaskEnables');
      | if strcmp(get_param(gcb, 'arith_type1'), 'Boolean'),
      | set_param(gcb, 'bitwidth1', '1');
      | set_param(gcb, 'bin_pt1', '0');
      | a(6) = {'off'};
      | a(8) = {'off'};
      | else
      | a(6) = {'on'};
      | a(8) = {'on'};
      | end
      | set_param(gcb, 'MaskEnables', a);
  fifoassign6_ : xbsIndex_r4/Slice  nbits=6  boolean_output=off  mode=Lower Bit Location + Width  bit1=0  base1=MSB of Input  bit0=4  base0=LSB of Input  dbl_ovrd=off  block_type=slice
  fifoassign6_1 : xbsIndex_r4/Slice  nbits=6  boolean_output=off  mode=Lower Bit Location + Width  bit1=0  base1=MSB of Input  bit0=10  base0=LSB of Input  dbl_ovrd=off  block_type=slice
  fifoassign6_2 : xbsIndex_r4/Slice  nbits=6  boolean_output=off  mode=Lower Bit Location + Width  bit1=0  base1=MSB of Input  bit0=16  base0=LSB of Input  dbl_ovrd=off  block_type=slice
  fifoassign6_3 : xbsIndex_r4/Slice  nbits=6  boolean_output=off  mode=Lower Bit Location + Width  bit1=0  base1=MSB of Input  bit0=22  base0=LSB of Input  dbl_ovrd=off  block_type=slice
  fix12_11_{,1..7} (8 alike) : xbsIndex_r4/Convert  gui_display_data_type=Fixed-point  arith_type="Signed  (2's comp)"  n_bits=12  bin_pt=11  float_type=Single  exp_bits=8  fraction_bits=24  quantization=Truncate  overflow=Saturate  en=off  latency=0  dbl_ovrd=off  pipeline=off  block_type=convert
  fsmph : Scope  NumInputPorts=8
      settings: YMin=-5~-5~-5~-5~-5~-5~-5~-5  YMax=5~5~5~5~5~5~5~5  SaveName=fsmdata
  fsmph1 : Scope  NumInputPorts=8
      settings: YMin=-5~-5~-5~-5~-5~-5~-5~-5  YMax=5~5~5~5~5~5~5~5  SaveName=fsmdata5
  gpio_a0 : xps_library/gpio  Tag=xps:gpio  io_group=ROACH:gpioa  io_dir=out  arith_type=Unsigned  bitwidth=1  bin_pt=0  bit_index=3  sample_period=1  use_single_ended=off  use_ddr=off  reg_iob=on  reg_clk_phase=0  termination=None
  gpio_a1 : xps_library/gpio  Tag=xps:gpio  io_group=ROACH:gpioa  io_dir=out  arith_type=Unsigned  bitwidth=1  bin_pt=0  bit_index=2  sample_period=1  use_single_ended=off  use_ddr=off  reg_iob=on  reg_clk_phase=0  termination=None
  gpio_a2 : xps_library/gpio  Tag=xps:gpio  io_group=ROACH:gpioa  io_dir=out  arith_type=Unsigned  bitwidth=1  bin_pt=0  bit_index=1  sample_period=1  use_single_ended=off  use_ddr=off  reg_iob=on  reg_clk_phase=0  termination=None
  gpio_a3 : xps_library/gpio  Tag=xps:gpio  io_group=ROACH:gpioa  io_dir=out  arith_type=Unsigned  bitwidth=1  bin_pt=0  bit_index=0  sample_period=1  use_single_ended=off  use_ddr=off  reg_iob=on  reg_clk_phase=0  termination=None
  gpio_a4 : xps_library/gpio  Tag=xps:gpio  io_group=ROACH:gpioa  io_dir=out  arith_type=Unsigned  bitwidth=1  bin_pt=0  bit_index=7  sample_period=1  use_single_ended=off  use_ddr=off  reg_iob=on  reg_clk_phase=0  termination=None
  gpio_a5 : xps_library/gpio  Tag=xps:gpio  io_group=ROACH:gpioa  io_dir=out  arith_type=Unsigned  bitwidth=1  bin_pt=0  bit_index=6  sample_period=1  use_single_ended=off  use_ddr=off  reg_iob=on  reg_clk_phase=0  termination=None
  holdcounter : Subsystem  Tag=xps:sw_reg  AncestorBlock=xps_library/software register  mask{numios=1, io_dir=From Processor, io_delay=0, sample_period=1, name1=reg, bitwidth1=32, arith_type1=Unsigned, bin_pt1=0}
      mask prompts: numios "Num I/Os"; io_dir "I/O direction"; io_delay "I/O delay"; sample_period "Sample period"; name1 "Name"; bitwidth1 "Bitwidth"; arith_type1 "Type"; bin_pt1 "Binary pt"
      mask init:
      | swreg_init(gcb);
      mask Callback numios: t = timer('StartDelay', 0.1); t.TimerFcn = {@swreg_cb, gcb}; start(t);
      mask TypeOptions io_dir: To Processor | From Processor
      mask Callback io_dir:
      | a = get_param(gcb, 'MaskEnables');
      | if strcmp(get_param(gcb, 'io_dir'), 'To Processor'),
      | a(4) = {'off'};
      | else
      | a(4) = {'on'};
      | end
      | set_param(gcb, 'MaskEnables', a);
      mask TypeOptions arith_type1: Unsigned | Signed  (2's comp) | Boolean
      mask Callback arith_type1:
      | a = get_param(gcb, 'MaskEnables');
      | if strcmp(get_param(gcb, 'arith_type1'), 'Boolean'),
      | set_param(gcb, 'bitwidth1', '1');
      | set_param(gcb, 'bin_pt1', '0');
      | a(6) = {'off'};
      | a(8) = {'off'};
      | else
      | a(6) = {'on'};
      | a(8) = {'on'};
      | end
      | set_param(gcb, 'MaskEnables', a);
  if_switch : Subsystem  Tag=xps:sw_reg  AncestorBlock=xps_library/software register  mask{numios=1, io_dir=From Processor, io_delay=0, sample_period=1, name1=reg, bitwidth1=32, arith_type1=Unsigned, bin_pt1=0}
      mask prompts: numios "Num I/Os"; io_dir "I/O direction"; io_delay "I/O delay"; sample_period "Sample period"; name1 "Name"; bitwidth1 "Bitwidth"; arith_type1 "Type"; bin_pt1 "Binary pt"
      mask init:
      | swreg_init(gcb);
      mask Callback numios: t = timer('StartDelay', 0.1); t.TimerFcn = {@swreg_cb, gcb}; start(t);
      mask TypeOptions io_dir: To Processor | From Processor
      mask Callback io_dir:
      | a = get_param(gcb, 'MaskEnables');
      | if strcmp(get_param(gcb, 'io_dir'), 'To Processor'),
      | a(4) = {'off'};
      | else
      | a(4) = {'on'};
      | end
      | set_param(gcb, 'MaskEnables', a);
      mask TypeOptions arith_type1: Unsigned | Signed  (2's comp) | Boolean
      mask Callback arith_type1:
      | a = get_param(gcb, 'MaskEnables');
      | if strcmp(get_param(gcb, 'arith_type1'), 'Boolean'),
      | set_param(gcb, 'bitwidth1', '1');
      | set_param(gcb, 'bin_pt1', '0');
      | a(6) = {'off'};
      | a(8) = {'off'};
      | else
      | a(6) = {'on'};
      | a(8) = {'on'};
      | end
      | set_param(gcb, 'MaskEnables', a);
  lastChanToRead : Subsystem  Tag=xps:sw_reg  AncestorBlock=xps_library/software register  mask{numios=1, io_dir=From Processor, io_delay=0, sample_period=1, name1=reg, bitwidth1=32, arith_type1=Unsigned, bin_pt1=0}
      mask prompts: numios "Num I/Os"; io_dir "I/O direction"; io_delay "I/O delay"; sample_period "Sample period"; name1 "Name"; bitwidth1 "Bitwidth"; arith_type1 "Type"; bin_pt1 "Binary pt"
      mask init:
      | swreg_init(gcb);
      mask Callback numios: t = timer('StartDelay', 0.1); t.TimerFcn = {@swreg_cb, gcb}; start(t);
      mask TypeOptions io_dir: To Processor | From Processor
      mask Callback io_dir:
      | a = get_param(gcb, 'MaskEnables');
      | if strcmp(get_param(gcb, 'io_dir'), 'To Processor'),
      | a(4) = {'off'};
      | else
      | a(4) = {'on'};
      | end
      | set_param(gcb, 'MaskEnables', a);
      mask TypeOptions arith_type1: Unsigned | Signed  (2's comp) | Boolean
      mask Callback arith_type1:
      | a = get_param(gcb, 'MaskEnables');
      | if strcmp(get_param(gcb, 'arith_type1'), 'Boolean'),
      | set_param(gcb, 'bitwidth1', '1');
      | set_param(gcb, 'bin_pt1', '0');
      | a(6) = {'off'};
      | a(8) = {'off'};
      | else
      | a(6) = {'on'};
      | a(8) = {'on'};
      | end
      | set_param(gcb, 'MaskEnables', a);
  low16_{0..7} (8 alike) : xbsIndex_r4/Slice  nbits=16  boolean_output=off  mode=Lower Bit Location + Width  bit1=0  base1=LSB of Input  bit0=0  base0=LSB of Input  dbl_ovrd=off  block_type=slice
  lsb0_5_1 : xbsIndex_r4/Slice  nbits=6  boolean_output=off  mode=Lower Bit Location + Width  bit1=0  base1=MSB of Input  bit0=0  base0=LSB of Input  dbl_ovrd=off  block_type=slice
  lsb8_ : xbsIndex_r4/Slice  nbits=8  boolean_output=off  mode=Lower Bit Location + Width  bit1=0  base1=MSB of Input  bit0=0  base0=LSB of Input  dbl_ovrd=off  block_type=slice
  maxNumBins : xbsIndex_r4/Constant  const=128  gui_display_data_type=Fixed-point  arith_type=Unsigned  n_bits=32  bin_pt=0  preci_type=Single  exp_width=8  frac_width=24  explicit_period=on  period=1  equ=P=C  opselect=C  inp2=PCIN>>17  opr=+  inp1=P  carry=CIN  dbl_ovrd=off  block_type=constant
  mux_en_nextstate : xbsIndex_r4/Mux  inputs=4  en=off  latency=0  precision=Full  arith_type=Unsigned  n_bits=16  bin_pt=14  quantization=Truncate  overflow=Wrap  dbl_ovrd=off  block_type=mux
  mux_output_fftsync : xbsIndex_r4/Mux  inputs=4  en=off  latency=0  precision=Full  arith_type=Unsigned  n_bits=16  bin_pt=14  quantization=Truncate  overflow=Wrap  dbl_ovrd=off  block_type=mux
  numffts : Subsystem  Tag=xps:sw_reg  AncestorBlock=xps_library/software register  mask{numios=1, io_dir=From Processor, io_delay=0, sample_period=1, name1=reg, bitwidth1=32, arith_type1=Unsigned, bin_pt1=0}
      mask prompts: numios "Num I/Os"; io_dir "I/O direction"; io_delay "I/O delay"; sample_period "Sample period"; name1 "Name"; bitwidth1 "Bitwidth"; arith_type1 "Type"; bin_pt1 "Binary pt"
      mask init:
      | swreg_init(gcb);
      mask Callback numios: t = timer('StartDelay', 0.1); t.TimerFcn = {@swreg_cb, gcb}; start(t);
      mask TypeOptions io_dir: To Processor | From Processor
      mask Callback io_dir:
      | a = get_param(gcb, 'MaskEnables');
      | if strcmp(get_param(gcb, 'io_dir'), 'To Processor'),
      | a(4) = {'off'};
      | else
      | a(4) = {'on'};
      | end
      | set_param(gcb, 'MaskEnables', a);
      mask TypeOptions arith_type1: Unsigned | Signed  (2's comp) | Boolean
      mask Callback arith_type1:
      | a = get_param(gcb, 'MaskEnables');
      | if strcmp(get_param(gcb, 'arith_type1'), 'Boolean'),
      | set_param(gcb, 'bitwidth1', '1');
      | set_param(gcb, 'bin_pt1', '0');
      | a(6) = {'off'};
      | a(8) = {'off'};
      | else
      | a(6) = {'on'};
      | a(8) = {'on'};
      | end
      | set_param(gcb, 'MaskEnables', a);
  outdata1 : Scope  NumInputPorts=4
      settings: YMin=-5~-5~-5~-5  YMax=5~5~5~5  SaveName=fsmdata8
  outmemscope : Scope  NumInputPorts=8
      settings: YMin=-5~-5~-5~-5~-5~-5~-5~-5  YMax=5~5~5~5~5~5~5~5  SaveName=fsmdata4
  overflowcounter : xbsIndex_r4/Counter  cnt_type=Free Running  cnt_to=Inf  operation=Up  start_count=0  cnt_by_val=1  arith_type=Unsigned  n_bits=32  bin_pt=0  load_pin=off  rst=on  en=on  explicit_period=on  period=1  dbl_ovrd=off  use_behavioral_HDL=off  implementation=Fabric  block_type=counter
  parallel_to_serial_converter1 : Subsystem  mask(parallel_to_serial_converter){pin_width=33, sout_width=1}
      mask prompts: pin_width "Parallel Input Width"; sout_width "Serial Output Width"
      mask help:
      | This block takes as input a parallel bus of specified width.
      | When the load signal 'ld' is asserted, this data is broken into
      | pieces of width specified by the serial output width and
      | stored into different registers chained to form a shift register.
      | If the 'shift' input is subsequently asserted, the shift register
      | returns as output a new piece of data of width sout_width.  This data
      | is the next least significant piece of the original bus.  The converter
      | serializes SMALL ENDIAN.
      |
      | Note that the load operation automatically loads the least significant
      | bits into the register closest to the output, so the first 'shift'
      | assertion changes the data output from bits [sout_width-1:0] to
      | bits [2*sout_width-1:sout_width].
      mask init:
      | parallel_to_serial_converter_init(gcb, ...
      |     'pin_width', pin_width, ...
      |     'sout_width', sout_width);
  pfb_fir : Subsystem  AncestorBlock=casper_library_pfbs/pfb_fir  mask(pfb_fir){PFBSize=9, TotalTaps=4, WindowType=hamming, n_inputs=2, MakeBiplex=off, BitWidthIn=12, BitWidthOut=12, CoeffBitWidth=12, CoeffDistMem=off, add_latency=1, mult_latency=2, bram_latency=2, fan_latency=1, quantization=Truncate, fwidth=1, mult_spec=2, coeffs_share=on}
      mask prompts: PFBSize "Size of PFB: (2^? pnts)"; TotalTaps "Total Number of Taps:"; WindowType "Windowing Function:"; n_inputs "Number of Simultaneous Inputs: (2^?)"; MakeBiplex "Make Biplex?"; BitWidthIn "Input Bitwidth:"; BitWidthOut "Output Bitwidth:"; CoeffBitWidth "Coefficient Bitwidth:"; CoeffDistMem "Use Distributed Memory for Coeffs"; add_latency "Add Latency"; mult_latency "Mult Latency"; bram_latency "BRAM Latency"; fan_latency "Fanout Latency"; quantization "Quantization Behavior"; fwidth "Bin Width Scaling (normal=1)"; mult_spec "Multiplier specification (0=core, 1=embedded, 2=behavioural) (left=1st tap, or just one value)"; coeffs_share "Share coefficients between polarisations (use less BRAM)?"
      mask init:
      | pfb_fir_init(gcb, ...
      |     'PFBSize', PFBSize, ...
      |     'TotalTaps', TotalTaps, ...
      |     'WindowType', WindowType, ...
      |     'n_inputs', n_inputs, ...
      |     'MakeBiplex', MakeBiplex, ...
      |     'BitWidthIn', BitWidthIn, ...
      |     'BitWidthOut', BitWidthOut, ...
      |     'CoeffBitWidth', CoeffBitWidth, ...
      |     'CoeffDistMem', CoeffDistMem, ...
      |     'add_latency', add_latency, ...
      |     'mult_latency', mult_latency, ...
      |     'bram_latency', bram_latency, ...
      |     'fan_latency', fan_latency, ...
      |     'quantization', quantization, ...
      |     'fwidth', fwidth, ...
      |     'mult_spec', mult_spec, ...
      |     'coeffs_share', coeffs_share);
      settings: AttributesFormatString=|
      | taps=4, add_latency=1
      | max scale 0.596
      mask Help: eval('xlWeb(''http://casper.berkeley.edu/wiki/Pfb_fir'')')
      mask Callback TotalTaps:
      | %num_taps = eval(get_param(gcb, 'TotalTaps'));
      | %old_vec = eval(get_param(gcb, 'mult_spec'));
      | 
      | %vec = 2.*ones(1,num_taps);
      | %old_size = length(old_vec);
      | 
      | %if(old_size <= num_taps),
      | %   new_size = old_size;
      | %else,
      | %    new_size = num_taps;
      | %end
      | 
      | %for n = 1:new_size, vec(n) = old_vec(n); end
      | %set_param(gcb, 'mult_spec', mat2str(vec));
      mask TypeOptions WindowType: bartlett | barthannwin | blackman | blackmanharris | bohamwin | chebwin | flattopwin | gausswin | hamming | hann | kaiser | nuttallwin | parzenwin | rectwin | tukeywin | triang | userwindow
      mask TypeOptions quantization: Truncate | Round  (unbiased: +/- Inf) | Round  (unbiased: Even Values)
      mask Callback fwidth:
      | %num_taps = eval(get_param(gcb, 'TotalTaps'));
      | %old_vec = eval(get_param(gcb, 'mult_spec'));
      | 
      | %vec = 2.*ones(1,num_taps);
      | %old_size = length(old_vec);
      | 
      | %if(old_size <= num_taps),
      | %    new_size = old_size;
      | %else,
      | %    new_size = num_taps;
      | %end
      | 
      | %for n = 1:new_size, vec(n) = old_vec(n); end
      | %set_param(gcb, 'mult_spec', mat2str(vec));
      mask Callback mult_spec:
      | %num_taps = eval(get_param(gcb, 'TotalTaps'));
      | %old_vec = eval(get_param(gcb, 'mult_spec'));
      | 
      | %vec = 2.*ones(1,num_taps);
      | %old_size = length(old_vec);
      | 
      | %if(old_size <= num_taps),
      | %    new_size = old_size;
      | %else,
      | %    new_size = num_taps;
      | %end
      | 
      | %for n = 1:new_size, vec(n) = old_vec(n); end
      | %set_param(gcb, 'mult_spec', mat2str(vec));
  pipeline : Subsystem  AncestorBlock=casper_library_delays/pipeline  mask(pipeline){latency=2}
      mask help:
      | An explicitly laid-out delay line to avoid mapping to SRL16s
      | for use in pipelining to help achieve timing closure.
      mask init:
      | pipeline_init(gcb,'latency',latency);
      settings: AttributesFormatString=Latency = %<latency>
      mask Display:
      | port_label('input', 1, 'd');
      | port_label('output', 1, 'q');
      | disp(['Z^-', num2str(latency)]);
  pipeline1 : Subsystem  AncestorBlock=casper_library_delays/pipeline  mask(pipeline){latency=2}
      mask help:
      | An explicitly laid-out delay line to avoid mapping to SRL16s
      | for use in pipelining to help achieve timing closure.
      mask init:
      | pipeline_init(gcb,'latency',latency);
      settings: AttributesFormatString=Latency = %<latency>
      mask Display:
      | port_label('input', 1, 'd');
      | port_label('output', 1, 'q');
      | disp(['Z^-', num2str(latency)]);
  pipeline2 : Subsystem  AncestorBlock=casper_library_delays/pipeline  mask(pipeline){latency=2}
      mask help:
      | An explicitly laid-out delay line to avoid mapping to SRL16s
      | for use in pipelining to help achieve timing closure.
      mask init:
      | pipeline_init(gcb,'latency',latency);
      settings: AttributesFormatString=Latency = %<latency>
      mask Display:
      | port_label('input', 1, 'd');
      | port_label('output', 1, 'q');
      | disp(['Z^-', num2str(latency)]);
  pipeline3 : Subsystem  AncestorBlock=casper_library_delays/pipeline  mask(pipeline){latency=2}
      mask help:
      | An explicitly laid-out delay line to avoid mapping to SRL16s
      | for use in pipelining to help achieve timing closure.
      mask init:
      | pipeline_init(gcb,'latency',latency);
      settings: AttributesFormatString=Latency = %<latency>
      mask Display:
      | port_label('input', 1, 'd');
      | port_label('output', 1, 'q');
      | disp(['Z^-', num2str(latency)]);
  pipeline4 : Subsystem  AncestorBlock=casper_library_delays/pipeline  mask(pipeline){latency=2}
      mask help:
      | An explicitly laid-out delay line to avoid mapping to SRL16s
      | for use in pipelining to help achieve timing closure.
      mask init:
      | pipeline_init(gcb,'latency',latency);
      settings: AttributesFormatString=Latency = %<latency>
      mask Display:
      | port_label('input', 1, 'd');
      | port_label('output', 1, 'q');
      | disp(['Z^-', num2str(latency)]);
  posedge1 : casper_library_misc/posedge  Tag=Rising Edge Detector
  posedge2 : Subsystem  Tag=Rising Edge Detector  mask(posedge){}
      mask help: Outputs true if a boolean input signal is true this clock and was false last clock.
      mask Help: eval('xlWeb([getenv(''MLIB_ROOT''), ''\doc\htmlblocks\sp_posedge\sp_posedge.html''])')
  posedge3 : casper_library_misc/posedge  Tag=Rising Edge Detector
  posedge5 : Subsystem  Tag=Rising Edge Detector  mask(posedge){}
      mask help: Outputs true if a boolean input signal is true this clock and was false last clock.
      mask Help: eval('xlWeb([getenv(''MLIB_ROOT''), ''\doc\htmlblocks\sp_posedge\sp_posedge.html''])')
  posedge6 : Subsystem  Tag=Rising Edge Detector  mask(posedge){}
      mask help: Outputs true if a boolean input signal is true this clock and was false last clock.
      mask Help: eval('xlWeb([getenv(''MLIB_ROOT''), ''\doc\htmlblocks\sp_posedge\sp_posedge.html''])')
  pulse_ext2 : casper_library_misc/pulse_ext  pulse_len=(34)*2^8
  pulse_ext3 : casper_library_misc/pulse_ext  pulse_len=(32)*2^8 + 2^7
  pulse_ext4 : casper_library_misc/pulse_ext  pulse_len=(18)*2^8 + 2^7
  pulse_ext5 : casper_library_misc/pulse_ext  pulse_len=(27)*2^8
  quartfull : xbsIndex_r4/Mux  inputs=4  en=off  latency=0  precision=Full  arith_type=Unsigned  n_bits=16  bin_pt=14  quantization=Truncate  overflow=Wrap  dbl_ovrd=off  block_type=mux
  readoutControl : Subsystem  Tag=xps:sw_reg  AncestorBlock=xps_library/software register  mask{numios=1, io_dir=From Processor, io_delay=0, sample_period=1, name1=reg, bitwidth1=32, arith_type1=Unsigned, bin_pt1=0}
      mask prompts: numios "Num I/Os"; io_dir "I/O direction"; io_delay "I/O delay"; sample_period "Sample period"; name1 "Name"; bitwidth1 "Bitwidth"; arith_type1 "Type"; bin_pt1 "Binary pt"
      mask init:
      | swreg_init(gcb);
      mask Callback numios: t = timer('StartDelay', 0.1); t.TimerFcn = {@swreg_cb, gcb}; start(t);
      mask TypeOptions io_dir: To Processor | From Processor
      mask Callback io_dir:
      | a = get_param(gcb, 'MaskEnables');
      | if strcmp(get_param(gcb, 'io_dir'), 'To Processor'),
      | a(4) = {'off'};
      | else
      | a(4) = {'on'};
      | end
      | set_param(gcb, 'MaskEnables', a);
      mask TypeOptions arith_type1: Unsigned | Signed  (2's comp) | Boolean
      mask Callback arith_type1:
      | a = get_param(gcb, 'MaskEnables');
      | if strcmp(get_param(gcb, 'arith_type1'), 'Boolean'),
      | set_param(gcb, 'bitwidth1', '1');
      | set_param(gcb, 'bin_pt1', '0');
      | a(6) = {'off'};
      | a(8) = {'off'};
      | else
      | a(6) = {'on'};
      | a(8) = {'on'};
      | end
      | set_param(gcb, 'MaskEnables', a);
  readoutStat : Subsystem  Tag=xps:sw_reg  AncestorBlock=xps_library/software register  mask{numios=1, io_dir=To Processor, io_delay=0, sample_period=1, name1=reg, bitwidth1=32, arith_type1=Unsigned, bin_pt1=0}
      mask prompts: numios "Num I/Os"; io_dir "I/O direction"; io_delay "I/O delay"; sample_period "Sample period"; name1 "Name"; bitwidth1 "Bitwidth"; arith_type1 "Type"; bin_pt1 "Binary pt"
      mask init:
      | swreg_init(gcb);
      mask Callback numios: t = timer('StartDelay', 0.1); t.TimerFcn = {@swreg_cb, gcb}; start(t);
      mask TypeOptions io_dir: To Processor | From Processor
      mask Callback io_dir:
      | a = get_param(gcb, 'MaskEnables');
      | if strcmp(get_param(gcb, 'io_dir'), 'To Processor'),
      | a(4) = {'off'};
      | else
      | a(4) = {'on'};
      | end
      | set_param(gcb, 'MaskEnables', a);
      mask TypeOptions arith_type1: Unsigned | Signed  (2's comp) | Boolean
      mask Callback arith_type1:
      | a = get_param(gcb, 'MaskEnables');
      | if strcmp(get_param(gcb, 'arith_type1'), 'Boolean'),
      | set_param(gcb, 'bitwidth1', '1');
      | set_param(gcb, 'bin_pt1', '0');
      | a(6) = {'off'};
      | a(8) = {'off'};
      | else
      | a(6) = {'on'};
      | a(8) = {'on'};
      | end
      | set_param(gcb, 'MaskEnables', a);
  regs : Subsystem  Tag=xps:sw_reg  AncestorBlock=xps_library/software register  mask{numios=1, io_dir=From Processor, io_delay=0, sample_period=1, name1=reg, bitwidth1=32, arith_type1=Unsigned, bin_pt1=0}
      mask prompts: numios "Num I/Os"; io_dir "I/O direction"; io_delay "I/O delay"; sample_period "Sample period"; name1 "Name"; bitwidth1 "Bitwidth"; arith_type1 "Type"; bin_pt1 "Binary pt"
      mask init:
      | swreg_init(gcb);
      mask Callback numios: t = timer('StartDelay', 0.1); t.TimerFcn = {@swreg_cb, gcb}; start(t);
      mask TypeOptions io_dir: To Processor | From Processor
      mask Callback io_dir:
      | a = get_param(gcb, 'MaskEnables');
      | if strcmp(get_param(gcb, 'io_dir'), 'To Processor'),
      | a(4) = {'off'};
      | else
      | a(4) = {'on'};
      | end
      | set_param(gcb, 'MaskEnables', a);
      mask TypeOptions arith_type1: Unsigned | Signed  (2's comp) | Boolean
      mask Callback arith_type1:
      | a = get_param(gcb, 'MaskEnables');
      | if strcmp(get_param(gcb, 'arith_type1'), 'Boolean'),
      | set_param(gcb, 'bitwidth1', '1');
      | set_param(gcb, 'bin_pt1', '0');
      | a(6) = {'off'};
      | a(8) = {'off'};
      | else
      | a(6) = {'on'};
      | a(8) = {'on'};
      | end
      | set_param(gcb, 'MaskEnables', a);
  rein_s_b15_{0..7} (8 alike) : xbsIndex_r4/Reinterpret  force_arith_type=on  arith_type="Signed  (2's comp)"  force_bin_pt=on  bin_pt=15  block_type=reinterpret
  resetDRAM : Subsystem  Tag=xps:sw_reg  AncestorBlock=xps_library/software register  mask{numios=1, io_dir=From Processor, io_delay=0, sample_period=1, name1=reg, bitwidth1=32, arith_type1=Unsigned, bin_pt1=0}
      mask prompts: numios "Num I/Os"; io_dir "I/O direction"; io_delay "I/O delay"; sample_period "Sample period"; name1 "Name"; bitwidth1 "Bitwidth"; arith_type1 "Type"; bin_pt1 "Binary pt"
      mask init:
      | swreg_init(gcb);
      mask Callback numios: t = timer('StartDelay', 0.1); t.TimerFcn = {@swreg_cb, gcb}; start(t);
      mask TypeOptions io_dir: To Processor | From Processor
      mask Callback io_dir:
      | a = get_param(gcb, 'MaskEnables');
      | if strcmp(get_param(gcb, 'io_dir'), 'To Processor'),
      | a(4) = {'off'};
      | else
      | a(4) = {'on'};
      | end
      | set_param(gcb, 'MaskEnables', a);
      mask TypeOptions arith_type1: Unsigned | Signed  (2's comp) | Boolean
      mask Callback arith_type1:
      | a = get_param(gcb, 'MaskEnables');
      | if strcmp(get_param(gcb, 'arith_type1'), 'Boolean'),
      | set_param(gcb, 'bitwidth1', '1');
      | set_param(gcb, 'bin_pt1', '0');
      | a(6) = {'off'};
      | a(8) = {'off'};
      | else
      | a(6) = {'on'};
      | a(8) = {'on'};
      | end
      | set_param(gcb, 'MaskEnables', a);
  restofbits_ : xbsIndex_r4/Constant  const=85  gui_display_data_type=Fixed-point  arith_type=Unsigned  n_bits=7  bin_pt=0  preci_type=Single  exp_width=8  frac_width=24  explicit_period=on  period=1  equ=P=C  opselect=C  inp2=PCIN>>17  opr=+  inp1=P  carry=CIN  dbl_ovrd=off  block_type=constant
  ri_to_c{,1..7} (8 alike) : casper_library_misc/ri_to_c
  savedEventCounter : Subsystem  Tag=xps:sw_reg  AncestorBlock=xps_library/software register  mask{numios=1, io_dir=To Processor, io_delay=0, sample_period=1, name1=reg, bitwidth1=32, arith_type1=Unsigned, bin_pt1=0}
      mask prompts: numios "Num I/Os"; io_dir "I/O direction"; io_delay "I/O delay"; sample_period "Sample period"; name1 "Name"; bitwidth1 "Bitwidth"; arith_type1 "Type"; bin_pt1 "Binary pt"
      mask init:
      | swreg_init(gcb);
      mask Callback numios: t = timer('StartDelay', 0.1); t.TimerFcn = {@swreg_cb, gcb}; start(t);
      mask TypeOptions io_dir: To Processor | From Processor
      mask Callback io_dir:
      | a = get_param(gcb, 'MaskEnables');
      | if strcmp(get_param(gcb, 'io_dir'), 'To Processor'),
      | a(4) = {'off'};
      | else
      | a(4) = {'on'};
      | end
      | set_param(gcb, 'MaskEnables', a);
      mask TypeOptions arith_type1: Unsigned | Signed  (2's comp) | Boolean
      mask Callback arith_type1:
      | a = get_param(gcb, 'MaskEnables');
      | if strcmp(get_param(gcb, 'arith_type1'), 'Boolean'),
      | set_param(gcb, 'bitwidth1', '1');
      | set_param(gcb, 'bin_pt1', '0');
      | a(6) = {'off'};
      | a(8) = {'off'};
      | else
      | a(6) = {'on'};
      | a(8) = {'on'};
      | end
      | set_param(gcb, 'MaskEnables', a);
  start : Subsystem  Tag=xps:sw_reg  AncestorBlock=xps_library/software register  mask{numios=1, io_dir=From Processor, io_delay=0, sample_period=1, name1=reg, bitwidth1=32, arith_type1=Unsigned, bin_pt1=0}
      mask prompts: numios "Num I/Os"; io_dir "I/O direction"; io_delay "I/O delay"; sample_period "Sample period"; name1 "Name"; bitwidth1 "Bitwidth"; arith_type1 "Type"; bin_pt1 "Binary pt"
      mask init:
      | swreg_init(gcb);
      mask Callback numios: t = timer('StartDelay', 0.1); t.TimerFcn = {@swreg_cb, gcb}; start(t);
      mask TypeOptions io_dir: To Processor | From Processor
      mask Callback io_dir:
      | a = get_param(gcb, 'MaskEnables');
      | if strcmp(get_param(gcb, 'io_dir'), 'To Processor'),
      | a(4) = {'off'};
      | else
      | a(4) = {'on'};
      | end
      | set_param(gcb, 'MaskEnables', a);
      mask TypeOptions arith_type1: Unsigned | Signed  (2's comp) | Boolean
      mask Callback arith_type1:
      | a = get_param(gcb, 'MaskEnables');
      | if strcmp(get_param(gcb, 'arith_type1'), 'Boolean'),
      | set_param(gcb, 'bitwidth1', '1');
      | set_param(gcb, 'bin_pt1', '0');
      | a(6) = {'off'};
      | a(8) = {'off'};
      | else
      | a(6) = {'on'};
      | a(8) = {'on'};
      | end
      | set_param(gcb, 'MaskEnables', a);
  statusFlags : Subsystem  Tag=xps:sw_reg  AncestorBlock=xps_library/software register  mask{numios=1, io_dir=To Processor, io_delay=0, sample_period=1, name1=reg, bitwidth1=32, arith_type1=Unsigned, bin_pt1=0}
      mask prompts: numios "Num I/Os"; io_dir "I/O direction"; io_delay "I/O delay"; sample_period "Sample period"; name1 "Name"; bitwidth1 "Bitwidth"; arith_type1 "Type"; bin_pt1 "Binary pt"
      mask init:
      | swreg_init(gcb);
      mask Callback numios: t = timer('StartDelay', 0.1); t.TimerFcn = {@swreg_cb, gcb}; start(t);
      mask TypeOptions io_dir: To Processor | From Processor
      mask Callback io_dir:
      | a = get_param(gcb, 'MaskEnables');
      | if strcmp(get_param(gcb, 'io_dir'), 'To Processor'),
      | a(4) = {'off'};
      | else
      | a(4) = {'on'};
      | end
      | set_param(gcb, 'MaskEnables', a);
      mask TypeOptions arith_type1: Unsigned | Signed  (2's comp) | Boolean
      mask Callback arith_type1:
      | a = get_param(gcb, 'MaskEnables');
      | if strcmp(get_param(gcb, 'arith_type1'), 'Boolean'),
      | set_param(gcb, 'bitwidth1', '1');
      | set_param(gcb, 'bin_pt1', '0');
      | a(6) = {'off'};
      | a(8) = {'off'};
      | else
      | a(6) = {'on'};
      | a(8) = {'on'};
      | end
      | set_param(gcb, 'MaskEnables', a);
  stb_en : Subsystem  Tag=xps:sw_reg  AncestorBlock=xps_library/software register  mask{numios=1, io_dir=From Processor, io_delay=0, sample_period=1, name1=reg, bitwidth1=32, arith_type1=Unsigned, bin_pt1=0}
      mask prompts: numios "Num I/Os"; io_dir "I/O direction"; io_delay "I/O delay"; sample_period "Sample period"; name1 "Name"; bitwidth1 "Bitwidth"; arith_type1 "Type"; bin_pt1 "Binary pt"
      mask init:
      | swreg_init(gcb);
      mask Callback numios: t = timer('StartDelay', 0.1); t.TimerFcn = {@swreg_cb, gcb}; start(t);
      mask TypeOptions io_dir: To Processor | From Processor
      mask Callback io_dir:
      | a = get_param(gcb, 'MaskEnables');
      | if strcmp(get_param(gcb, 'io_dir'), 'To Processor'),
      | a(4) = {'off'};
      | else
      | a(4) = {'on'};
      | end
      | set_param(gcb, 'MaskEnables', a);
      mask TypeOptions arith_type1: Unsigned | Signed  (2's comp) | Boolean
      mask Callback arith_type1:
      | a = get_param(gcb, 'MaskEnables');
      | if strcmp(get_param(gcb, 'arith_type1'), 'Boolean'),
      | set_param(gcb, 'bitwidth1', '1');
      | set_param(gcb, 'bin_pt1', '0');
      | a(6) = {'off'};
      | a(8) = {'off'};
      | else
      | a(6) = {'on'};
      | a(8) = {'on'};
      | end
      | set_param(gcb, 'MaskEnables', a);
  stffts_fsm : Subsystem  Tag=xps:sw_reg  AncestorBlock=xps_library/software register  mask{numios=1, io_dir=To Processor, io_delay=0, sample_period=1, name1=reg, bitwidth1=32, arith_type1=Unsigned, bin_pt1=0}
      mask prompts: numios "Num I/Os"; io_dir "I/O direction"; io_delay "I/O delay"; sample_period "Sample period"; name1 "Name"; bitwidth1 "Bitwidth"; arith_type1 "Type"; bin_pt1 "Binary pt"
      mask init:
      | swreg_init(gcb);
      mask Callback numios: t = timer('StartDelay', 0.1); t.TimerFcn = {@swreg_cb, gcb}; start(t);
      mask TypeOptions io_dir: To Processor | From Processor
      mask Callback io_dir:
      | a = get_param(gcb, 'MaskEnables');
      | if strcmp(get_param(gcb, 'io_dir'), 'To Processor'),
      | a(4) = {'off'};
      | else
      | a(4) = {'on'};
      | end
      | set_param(gcb, 'MaskEnables', a);
      mask TypeOptions arith_type1: Unsigned | Signed  (2's comp) | Boolean
      mask Callback arith_type1:
      | a = get_param(gcb, 'MaskEnables');
      | if strcmp(get_param(gcb, 'arith_type1'), 'Boolean'),
      | set_param(gcb, 'bitwidth1', '1');
      | set_param(gcb, 'bin_pt1', '0');
      | a(6) = {'off'};
      | a(8) = {'off'};
      | else
      | a(6) = {'on'};
      | a(8) = {'on'};
      | end
      | set_param(gcb, 'MaskEnables', a);
  testFreq : Subsystem  Tag=xps:sw_reg  AncestorBlock=xps_library/software register  mask{numios=1, io_dir=From Processor, io_delay=0, sample_period=1, name1=reg, bitwidth1=32, arith_type1=Unsigned, bin_pt1=0}
      mask prompts: numios "Num I/Os"; io_dir "I/O direction"; io_delay "I/O delay"; sample_period "Sample period"; name1 "Name"; bitwidth1 "Bitwidth"; arith_type1 "Type"; bin_pt1 "Binary pt"
      mask init:
      | swreg_init(gcb);
      mask Callback numios: t = timer('StartDelay', 0.1); t.TimerFcn = {@swreg_cb, gcb}; start(t);
      mask TypeOptions io_dir: To Processor | From Processor
      mask Callback io_dir:
      | a = get_param(gcb, 'MaskEnables');
      | if strcmp(get_param(gcb, 'io_dir'), 'To Processor'),
      | a(4) = {'off'};
      | else
      | a(4) = {'on'};
      | end
      | set_param(gcb, 'MaskEnables', a);
      mask TypeOptions arith_type1: Unsigned | Signed  (2's comp) | Boolean
      mask Callback arith_type1:
      | a = get_param(gcb, 'MaskEnables');
      | if strcmp(get_param(gcb, 'arith_type1'), 'Boolean'),
      | set_param(gcb, 'bitwidth1', '1');
      | set_param(gcb, 'bin_pt1', '0');
      | a(6) = {'off'};
      | a(8) = {'off'};
      | else
      | a(6) = {'on'};
      | a(8) = {'on'};
      | end
      | set_param(gcb, 'MaskEnables', a);
  testFreq1 : Subsystem  Tag=xps:sw_reg  AncestorBlock=xps_library/software register  mask{numios=1, io_dir=From Processor, io_delay=0, sample_period=1, name1=reg, bitwidth1=32, arith_type1=Unsigned, bin_pt1=0}
      mask prompts: numios "Num I/Os"; io_dir "I/O direction"; io_delay "I/O delay"; sample_period "Sample period"; name1 "Name"; bitwidth1 "Bitwidth"; arith_type1 "Type"; bin_pt1 "Binary pt"
      mask init:
      | swreg_init(gcb);
      mask Callback numios: t = timer('StartDelay', 0.1); t.TimerFcn = {@swreg_cb, gcb}; start(t);
      mask TypeOptions io_dir: To Processor | From Processor
      mask Callback io_dir:
      | a = get_param(gcb, 'MaskEnables');
      | if strcmp(get_param(gcb, 'io_dir'), 'To Processor'),
      | a(4) = {'off'};
      | else
      | a(4) = {'on'};
      | end
      | set_param(gcb, 'MaskEnables', a);
      mask TypeOptions arith_type1: Unsigned | Signed  (2's comp) | Boolean
      mask Callback arith_type1:
      | a = get_param(gcb, 'MaskEnables');
      | if strcmp(get_param(gcb, 'arith_type1'), 'Boolean'),
      | set_param(gcb, 'bitwidth1', '1');
      | set_param(gcb, 'bin_pt1', '0');
      | a(6) = {'off'};
      | a(8) = {'off'};
      | else
      | a(6) = {'on'};
      | a(8) = {'on'};
      | end
      | set_param(gcb, 'MaskEnables', a);
  testFreq2 : Subsystem  Tag=xps:sw_reg  AncestorBlock=xps_library/software register  mask{numios=1, io_dir=From Processor, io_delay=0, sample_period=1, name1=reg, bitwidth1=32, arith_type1=Unsigned, bin_pt1=0}
      mask prompts: numios "Num I/Os"; io_dir "I/O direction"; io_delay "I/O delay"; sample_period "Sample period"; name1 "Name"; bitwidth1 "Bitwidth"; arith_type1 "Type"; bin_pt1 "Binary pt"
      mask init:
      | swreg_init(gcb);
      mask Callback numios: t = timer('StartDelay', 0.1); t.TimerFcn = {@swreg_cb, gcb}; start(t);
      mask TypeOptions io_dir: To Processor | From Processor
      mask Callback io_dir:
      | a = get_param(gcb, 'MaskEnables');
      | if strcmp(get_param(gcb, 'io_dir'), 'To Processor'),
      | a(4) = {'off'};
      | else
      | a(4) = {'on'};
      | end
      | set_param(gcb, 'MaskEnables', a);
      mask TypeOptions arith_type1: Unsigned | Signed  (2's comp) | Boolean
      mask Callback arith_type1:
      | a = get_param(gcb, 'MaskEnables');
      | if strcmp(get_param(gcb, 'arith_type1'), 'Boolean'),
      | set_param(gcb, 'bitwidth1', '1');
      | set_param(gcb, 'bin_pt1', '0');
      | a(6) = {'off'};
      | a(8) = {'off'};
      | else
      | a(6) = {'on'};
      | a(8) = {'on'};
      | end
      | set_param(gcb, 'MaskEnables', a);
  testFreq3 : Subsystem  Tag=xps:sw_reg  AncestorBlock=xps_library/software register  mask{numios=1, io_dir=From Processor, io_delay=0, sample_period=1, name1=reg, bitwidth1=32, arith_type1=Unsigned, bin_pt1=0}
      mask prompts: numios "Num I/Os"; io_dir "I/O direction"; io_delay "I/O delay"; sample_period "Sample period"; name1 "Name"; bitwidth1 "Bitwidth"; arith_type1 "Type"; bin_pt1 "Binary pt"
      mask init:
      | swreg_init(gcb);
      mask Callback numios: t = timer('StartDelay', 0.1); t.TimerFcn = {@swreg_cb, gcb}; start(t);
      mask TypeOptions io_dir: To Processor | From Processor
      mask Callback io_dir:
      | a = get_param(gcb, 'MaskEnables');
      | if strcmp(get_param(gcb, 'io_dir'), 'To Processor'),
      | a(4) = {'off'};
      | else
      | a(4) = {'on'};
      | end
      | set_param(gcb, 'MaskEnables', a);
      mask TypeOptions arith_type1: Unsigned | Signed  (2's comp) | Boolean
      mask Callback arith_type1:
      | a = get_param(gcb, 'MaskEnables');
      | if strcmp(get_param(gcb, 'arith_type1'), 'Boolean'),
      | set_param(gcb, 'bitwidth1', '1');
      | set_param(gcb, 'bin_pt1', '0');
      | a(6) = {'off'};
      | a(8) = {'off'};
      | else
      | a(6) = {'on'};
      | a(8) = {'on'};
      | end
      | set_param(gcb, 'MaskEnables', a);
  testFreq4 : Subsystem  Tag=xps:sw_reg  AncestorBlock=xps_library/software register  mask{numios=1, io_dir=From Processor, io_delay=0, sample_period=1, name1=reg, bitwidth1=32, arith_type1=Unsigned, bin_pt1=0}
      mask prompts: numios "Num I/Os"; io_dir "I/O direction"; io_delay "I/O delay"; sample_period "Sample period"; name1 "Name"; bitwidth1 "Bitwidth"; arith_type1 "Type"; bin_pt1 "Binary pt"
      mask init:
      | swreg_init(gcb);
      mask Callback numios: t = timer('StartDelay', 0.1); t.TimerFcn = {@swreg_cb, gcb}; start(t);
      mask TypeOptions io_dir: To Processor | From Processor
      mask Callback io_dir:
      | a = get_param(gcb, 'MaskEnables');
      | if strcmp(get_param(gcb, 'io_dir'), 'To Processor'),
      | a(4) = {'off'};
      | else
      | a(4) = {'on'};
      | end
      | set_param(gcb, 'MaskEnables', a);
      mask TypeOptions arith_type1: Unsigned | Signed  (2's comp) | Boolean
      mask Callback arith_type1:
      | a = get_param(gcb, 'MaskEnables');
      | if strcmp(get_param(gcb, 'arith_type1'), 'Boolean'),
      | set_param(gcb, 'bitwidth1', '1');
      | set_param(gcb, 'bin_pt1', '0');
      | a(6) = {'off'};
      | a(8) = {'off'};
      | else
      | a(6) = {'on'};
      | a(8) = {'on'};
      | end
      | set_param(gcb, 'MaskEnables', a);
  testFreq5 : Subsystem  Tag=xps:sw_reg  AncestorBlock=xps_library/software register  mask{numios=1, io_dir=From Processor, io_delay=0, sample_period=1, name1=reg, bitwidth1=32, arith_type1=Unsigned, bin_pt1=0}
      mask prompts: numios "Num I/Os"; io_dir "I/O direction"; io_delay "I/O delay"; sample_period "Sample period"; name1 "Name"; bitwidth1 "Bitwidth"; arith_type1 "Type"; bin_pt1 "Binary pt"
      mask init:
      | swreg_init(gcb);
      mask Callback numios: t = timer('StartDelay', 0.1); t.TimerFcn = {@swreg_cb, gcb}; start(t);
      mask TypeOptions io_dir: To Processor | From Processor
      mask Callback io_dir:
      | a = get_param(gcb, 'MaskEnables');
      | if strcmp(get_param(gcb, 'io_dir'), 'To Processor'),
      | a(4) = {'off'};
      | else
      | a(4) = {'on'};
      | end
      | set_param(gcb, 'MaskEnables', a);
      mask TypeOptions arith_type1: Unsigned | Signed  (2's comp) | Boolean
      mask Callback arith_type1:
      | a = get_param(gcb, 'MaskEnables');
      | if strcmp(get_param(gcb, 'arith_type1'), 'Boolean'),
      | set_param(gcb, 'bitwidth1', '1');
      | set_param(gcb, 'bin_pt1', '0');
      | a(6) = {'off'};
      | a(8) = {'off'};
      | else
      | a(6) = {'on'};
      | a(8) = {'on'};
      | end
      | set_param(gcb, 'MaskEnables', a);
  testFreq6 : Subsystem  Tag=xps:sw_reg  AncestorBlock=xps_library/software register  mask{numios=1, io_dir=From Processor, io_delay=0, sample_period=1, name1=reg, bitwidth1=32, arith_type1=Unsigned, bin_pt1=0}
      mask prompts: numios "Num I/Os"; io_dir "I/O direction"; io_delay "I/O delay"; sample_period "Sample period"; name1 "Name"; bitwidth1 "Bitwidth"; arith_type1 "Type"; bin_pt1 "Binary pt"
      mask init:
      | swreg_init(gcb);
      mask Callback numios: t = timer('StartDelay', 0.1); t.TimerFcn = {@swreg_cb, gcb}; start(t);
      mask TypeOptions io_dir: To Processor | From Processor
      mask Callback io_dir:
      | a = get_param(gcb, 'MaskEnables');
      | if strcmp(get_param(gcb, 'io_dir'), 'To Processor'),
      | a(4) = {'off'};
      | else
      | a(4) = {'on'};
      | end
      | set_param(gcb, 'MaskEnables', a);
      mask TypeOptions arith_type1: Unsigned | Signed  (2's comp) | Boolean
      mask Callback arith_type1:
      | a = get_param(gcb, 'MaskEnables');
      | if strcmp(get_param(gcb, 'arith_type1'), 'Boolean'),
      | set_param(gcb, 'bitwidth1', '1');
      | set_param(gcb, 'bin_pt1', '0');
      | a(6) = {'off'};
      | a(8) = {'off'};
      | else
      | a(6) = {'on'};
      | a(8) = {'on'};
      | end
      | set_param(gcb, 'MaskEnables', a);
  testFreq7 : Subsystem  Tag=xps:sw_reg  AncestorBlock=xps_library/software register  mask{numios=1, io_dir=From Processor, io_delay=0, sample_period=1, name1=reg, bitwidth1=32, arith_type1=Unsigned, bin_pt1=0}
      mask prompts: numios "Num I/Os"; io_dir "I/O direction"; io_delay "I/O delay"; sample_period "Sample period"; name1 "Name"; bitwidth1 "Bitwidth"; arith_type1 "Type"; bin_pt1 "Binary pt"
      mask init:
      | swreg_init(gcb);
      mask Callback numios: t = timer('StartDelay', 0.1); t.TimerFcn = {@swreg_cb, gcb}; start(t);
      mask TypeOptions io_dir: To Processor | From Processor
      mask Callback io_dir:
      | a = get_param(gcb, 'MaskEnables');
      | if strcmp(get_param(gcb, 'io_dir'), 'To Processor'),
      | a(4) = {'off'};
      | else
      | a(4) = {'on'};
      | end
      | set_param(gcb, 'MaskEnables', a);
      mask TypeOptions arith_type1: Unsigned | Signed  (2's comp) | Boolean
      mask Callback arith_type1:
      | a = get_param(gcb, 'MaskEnables');
      | if strcmp(get_param(gcb, 'arith_type1'), 'Boolean'),
      | set_param(gcb, 'bitwidth1', '1');
      | set_param(gcb, 'bin_pt1', '0');
      | a(6) = {'off'};
      | a(8) = {'off'};
      | else
      | a(6) = {'on'};
      | a(8) = {'on'};
      | end
      | set_param(gcb, 'MaskEnables', a);
  timestamp_out : Subsystem  Tag=xps:sw_reg  AncestorBlock=xps_library/software register  mask{numios=1, io_dir=To Processor, io_delay=0, sample_period=1, name1=reg, bitwidth1=32, arith_type1=Unsigned, bin_pt1=0}
      mask prompts: numios "Num I/Os"; io_dir "I/O direction"; io_delay "I/O delay"; sample_period "Sample period"; name1 "Name"; bitwidth1 "Bitwidth"; arith_type1 "Type"; bin_pt1 "Binary pt"
      mask init:
      | swreg_init(gcb);
      mask Callback numios: t = timer('StartDelay', 0.1); t.TimerFcn = {@swreg_cb, gcb}; start(t);
      mask TypeOptions io_dir: To Processor | From Processor
      mask Callback io_dir:
      | a = get_param(gcb, 'MaskEnables');
      | if strcmp(get_param(gcb, 'io_dir'), 'To Processor'),
      | a(4) = {'off'};
      | else
      | a(4) = {'on'};
      | end
      | set_param(gcb, 'MaskEnables', a);
      mask TypeOptions arith_type1: Unsigned | Signed  (2's comp) | Boolean
      mask Callback arith_type1:
      | a = get_param(gcb, 'MaskEnables');
      | if strcmp(get_param(gcb, 'arith_type1'), 'Boolean'),
      | set_param(gcb, 'bitwidth1', '1');
      | set_param(gcb, 'bin_pt1', '0');
      | a(6) = {'off'};
      | a(8) = {'off'};
      | else
      | a(6) = {'on'};
      | a(8) = {'on'};
      | end
      | set_param(gcb, 'MaskEnables', a);
  timestamper : xbsIndex_r4/Counter  cnt_type=Free Running  cnt_to=Inf  operation=Up  start_count=0  cnt_by_val=1  arith_type=Unsigned  n_bits=32  bin_pt=0  load_pin=off  rst=on  en=on  explicit_period=on  period=1  dbl_ovrd=off  use_behavioral_HDL=off  implementation=Fabric  block_type=counter
  ui16_1 : xbsIndex_r4/Constant  const=43690  gui_display_data_type=Fixed-point  arith_type=Unsigned  n_bits=16  bin_pt=0  preci_type=Single  exp_width=8  frac_width=24  explicit_period=on  period=1  equ=P=C  opselect=C  inp2=PCIN>>17  opr=+  inp1=P  carry=CIN  dbl_ovrd=off  block_type=constant
  ui16_10 : xbsIndex_r4/Reinterpret  force_arith_type=on  arith_type=Unsigned  force_bin_pt=on  bin_pt=0  block_type=reinterpret
  ui16_2 : xbsIndex_r4/Reinterpret  force_arith_type=on  arith_type=Unsigned  force_bin_pt=on  bin_pt=0  block_type=reinterpret
  ui32_ : xbsIndex_r4/Constant  const=0  gui_display_data_type=Fixed-point  arith_type=Unsigned  n_bits=32  bin_pt=0  preci_type=Single  exp_width=8  frac_width=24  explicit_period=on  period=1  equ=P=C  opselect=C  inp2=PCIN>>17  opr=+  inp1=P  carry=CIN  dbl_ovrd=off  block_type=constant
  vldmux : xbsIndex_r4/Mux  inputs=4  en=off  latency=0  precision=Full  arith_type=Unsigned  n_bits=16  bin_pt=14  quantization=Truncate  overflow=Wrap  dbl_ovrd=off  block_type=mux
  wr_coef{0..3} (4 alike) : xbsIndex_r4/Logical  logical_function=AND  inputs=2  en=off  latency=0  precision=Full  arith_type=Unsigned  n_bits=16  bin_pt=0  align_bp=on  dbl_ovrd=off  block_type=logical
  zero_bool_{1..4} (4 alike) : xbsIndex_r4/Constant  const=1  gui_display_data_type=Boolean  arith_type=Boolean  n_bits=36  bin_pt=0  preci_type=Single  exp_width=8  frac_width=24  explicit_period=on  period=1  equ=P=C  opselect=C  inp2=PCIN>>17  opr=+  inp1=P  carry=CIN  dbl_ovrd=off  block_type=constant
  zero_bool_5 : xbsIndex_r4/Constant  const=0  gui_display_data_type=Boolean  arith_type=Boolean  n_bits=36  bin_pt=0  preci_type=Single  exp_width=8  frac_width=24  explicit_period=on  period=1  equ=P=C  opselect=C  inp2=PCIN>>17  opr=+  inp1=P  carry=CIN  dbl_ovrd=off  block_type=constant
  zero_bool_6 : xbsIndex_r4/Constant  const=0  gui_display_data_type=Boolean  arith_type=Boolean  n_bits=36  bin_pt=0  preci_type=Single  exp_width=8  frac_width=24  explicit_period=on  period=1  equ=P=C  opselect=C  inp2=PCIN>>17  opr=+  inp1=P  carry=CIN  dbl_ovrd=off  block_type=constant
  wires:
  Constant6/1 -> dac_mkid_4x/11
  Constant8/1 -> dac_mkid_4x/12
  Convert5/1 -> parallel_to_serial_converter1/1(pin)
  Constant11/1 -> stb_en/1(sim_reg)
  Pulse Generator2/1 -> start/1(sim_reg)
  stb_en/1(in_reg) -> Slice15/1
  Slice14/1 -> Logical8/2
  SWAT_LE/1(in_reg) -> Slice14/1
  Inverter3/1 -> Delay28/1
  Logical8/1 -> Inverter3/1
  pulse_ext4/1 -> Logical8/1
  Slice21/1 -> Logical7/2
  Inverter1/1 -> Delay27/1
  Logical7/1 -> Inverter1/1
  LO_SLE/1(in_reg) -> Slice21/1
  pulse_ext3/1 -> Logical7/1
  Constant12/1 -> SER_DI/1(sim_reg)
  posedge6/1(Out) -> parallel_to_serial_converter1/3(shift)
  Slice26/1 -> posedge2/1(In)
  Inverter5/1 -> Counter2/1
  Counter2/1 -> Slice3/1
  Slice3/1 -> posedge6/1(In), Delay24/1
  Logical9/1 -> Delay23/1
  Counter4/1 -> Slice10/1
  Slice10/1 -> Logical9/2
  pulse_ext5/1 -> Inverter2/1
  Inverter2/1 -> Logical9/3
  Constant14/1 -> LO_SLE/1(sim_reg)
  Constant15/1 -> SWAT_LE/1(sim_reg)
  Inverter4/1 -> Counter4/1
  start/1(in_reg) -> Slice26/1
  posedge2/1(Out) -> pulse_ext2/1
  pulse_ext2/1 -> Counter2/2, Counter4/2, Inverter4/1, Inverter5/1, posedge5/1(In)
  posedge5/1(Out) -> parallel_to_serial_converter1/2(ld), pulse_ext5/1, pulse_ext3/1, pulse_ext4/1
  Delay23/1 -> Mux2/2
  Mux2/1 -> Delay34/1
  parallel_to_serial_converter1/1(sout) -> Mux3/2
  Mux3/1 -> Delay30/1
  Delay28/1 -> Mux4/2
  Mux4/1 -> Delay32/1
  Delay27/1 -> Mux5/2
  Delay24/1 -> Mux6/2
  Mux6/1 -> Delay29/1
  Mux5/1 -> Delay31/1
  From Workspace1/1 -> if_switch/1(sim_reg)
  if_switch/1(in_reg) -> Slice2/1
  Slice2/1 -> [if_switch]
  [if_switch] -> Mux2/1
  [if_switch] -> Mux6/1
  [if_switch] -> Mux3/1
  [if_switch] -> Mux5/1
  [if_switch] -> Mux4/1
  From Workspace2/1 -> regs/1(sim_reg)
  regs/1(in_reg) -> Slice20/1, Slice22/1, Slice25/1, Slice11/1, Slice4/1, Slice1/1
  Slice22/1 -> [ser_clk]
  Slice20/1 -> [sw_stb]
  Slice25/1 -> [ser_di]
  Slice11/1 -> [lo_sle]
  Slice1/1 -> [swat_le]
  [sw_stb] -> Mux2/3
  [ser_clk] -> Mux6/3
  [ser_di] -> Mux3/3
  [lo_sle] -> Mux5/3
  [swat_le] -> Mux4/3
  Delay34/1 -> gpio_a0/1
  Delay29/1 -> gpio_a1/1
  Delay30/1 -> gpio_a2/1
  Delay31/1 -> gpio_a3/1
  Delay32/1 -> gpio_a5/1
  SER_DI/1(in_reg) -> Convert5/1
  Slice15/1 -> Logical9/1
  gpio_a0/1 -> Terminator/1
  gpio_a1/1 -> Terminator3/1
  gpio_a2/1 -> Terminator4/1
  gpio_a3/1 -> Terminator5/1
  gpio_a5/1 -> Terminator6/1
  Slice4/1 -> [clk_sle]
  gpio_a4/1 -> Terminator7/1
  [clk_sle] -> gpio_a4/1
  [startDac] -> dac_mkid_4x/9, dac_mkid_4x/10
  Mux9/1 -> [adc_q0]
  Mux1/1 -> [adc_i1]
  Mux10/1 -> [adc_q1]
  Mux7/1 -> [adc_i2]
  Mux8/1 -> [adc_i3]
  Logical17/1 -> [adcvalid]
  adcWaveMem/1(Out1) -> [adcwavememDone]
  [adcwavememStart] -> adcWaveMem/1(Start)
  adc_mkid_4x/9 -> Logical17/1
  [adcforcesync] -> Logical17/2
  adc_mkid_4x/1 -> Mux/3
  adc_mkid_4x/2 -> Mux1/3
  adc_mkid_4x/3 -> Mux7/3
  adc_mkid_4x/4 -> Mux8/3
  adc_mkid_4x/5 -> Mux9/3
  adc_mkid_4x/6 -> Mux10/3
  adc_mkid_4x/7 -> Mux11/3
  adc_mkid_4x/8 -> Mux12/3
  [dacLoopBack] -> Mux/1
  [dacLoopBack] -> Mux1/1
  [dacLoopBack] -> Mux7/1
  [dacLoopBack] -> Mux8/1
  [dacLoopBack] -> Mux9/1
  [dacLoopBack] -> Mux10/1
  [dacLoopBack] -> Mux11/1
  [dacLoopBack] -> Mux12/1
  [daci0] -> fix12_11_/1
  [daci1] -> fix12_11_1/1
  [daci2] -> fix12_11_2/1
  [daci3] -> fix12_11_4/1
  [dacq0] -> fix12_11_3/1
  [dacq1] -> fix12_11_5/1
  [dacq2] -> fix12_11_6/1
  [dacq3] -> fix12_11_7/1
  fix12_11_/1 -> Mux/2
  fix12_11_1/1 -> Mux1/2
  fix12_11_2/1 -> Mux7/2
  fix12_11_4/1 -> Mux8/2
  fix12_11_3/1 -> Mux9/2
  fix12_11_5/1 -> Mux10/2
  fix12_11_6/1 -> Mux11/2
  fix12_11_7/1 -> Mux12/2
  Mux/1 -> [adc_i0]
  Mux11/1 -> [adc_q2]
  Mux12/1 -> [adc_q3]
  [adc_i0] -> adcWaveMem/3(Src0)
  Constant/1 -> adcWaveMem/6(WE1)
  [adcwavememSel] -> adcWaveMem/2(Sel)
  [adc_i1] -> adcWaveMem/4(Src1)
  [adcwavememWE] -> adcWaveMem/5(WE)
  [LUTsize] -> DRAM_LUT/1(LUTsize)
  resetDRAM/1(in_reg) -> Slice13/1
  From Workspace7/1 -> resetDRAM/1(sim_reg)
  Slice13/1 -> DRAM_LUT/4(resetDRAM)
  RWen/1(in_reg) -> Slice23/1
  From Workspace8/1 -> RWen/1(sim_reg)
  Slice23/1 -> DRAM_LUT/5(RWen)
  holdcounter/1(in_reg) -> Slice24/1
  From Workspace9/1 -> holdcounter/1(sim_reg)
  Slice24/1 -> DRAM_LUT/6(holdcounter)
  DRAM_LUT/2(data_i1) -> Mux14/2, dac_mkid_4x/2
  DRAM_LUT/3(data_i2) -> dac_mkid_4x/3, Mux15/2
  DRAM_LUT/4(data_i3) -> dac_mkid_4x/4, Mux16/2
  DRAM_LUT/5(data_q0) -> Mux17/2, dac_mkid_4x/5
  DRAM_LUT/6(data_q1) -> dac_mkid_4x/6, Mux18/2
  DRAM_LUT/7(data_q2) -> dac_mkid_4x/7, Mux19/2
  DRAM_LUT/8(data_q3) -> Mux20/2, dac_mkid_4x/8
  From Workspace10/1 -> LUTsize/1(sim_reg)
  [seeaddress] -> DRAM_LUT/7(seeaddress)
  Delay9/1 -> pfb_fir/2(pol1_in1)
  Delay10/1 -> pfb_fir/3(pol1_in2)
  Delay11/1 -> pfb_fir/4(pol1_in3)
  Delay12/1 -> pfb_fir/5(pol1_in4)
  ri_to_c3/1 -> Delay12/1
  ri_to_c2/1 -> Delay11/1
  ri_to_c1/1 -> Delay10/1
  ri_to_c/1 -> Delay9/1
  pfb_fir/5(pol1_out4) -> pipeline4/1(d)
  pfb_fir/4(pol1_out3) -> pipeline3/1(d)
  pfb_fir/3(pol1_out2) -> pipeline2/1(d)
  pfb_fir/2(pol1_out1) -> pipeline1/1(d)
  pfb_fir/1(sync_out) -> pipeline/1(d)
  pipeline/1(q) -> fft1/1(sync)
  [fftmask] -> fft1/2(shift)
  [adc_q0] -> Delay1/1
  [adc_i0] -> Delay3/1
  Delay13/1 -> c2polar_1/1(c), [fftcoef0]
  Delay14/1 -> c2polar_2/1(c), [fftcoef1]
  Delay15/1 -> c2polar_3/1(c), [fftcoef2]
  Delay16/1 -> c2polar_5/1(c), [fftcoef3]
  fft1/2(out00) -> Delay13/1
  fft1/3(out01) -> Delay14/1
  fft1/4(out02) -> Delay15/1
  fft1/5(out03) -> Delay16/1
  fft1/1(sync_out) -> [fftsyncout]
  [adc_q1] -> Delay5/1
  [adc_i1] -> Delay4/1
  [adc_q2] -> Delay7/1
  [adc_i2] -> Delay6/1
  [adc_q3] -> Delay17/1
  [adc_i3] -> Delay8/1
  Delay3/1 -> ri_to_c/1
  Delay1/1 -> ri_to_c/2
  Delay4/1 -> ri_to_c1/1
  Delay5/1 -> ri_to_c1/2
  Delay6/1 -> ri_to_c2/1
  Delay7/1 -> ri_to_c2/2
  Delay17/1 -> ri_to_c3/2
  Delay8/1 -> ri_to_c3/1
  Convert4/1 -> Reinterpret1/1
  Convert9/1 -> Reinterpret5/1
  c_to_ri/2 -> Convert4/1
  c_to_ri/1 -> Convert9/1
  Reinterpret5/1 -> ri_to_c4/1
  Reinterpret1/1 -> ri_to_c4/2
  Convert6/1 -> Reinterpret2/1
  Convert7/1 -> Reinterpret3/1
  c_to_ri1/2 -> Convert6/1
  c_to_ri1/1 -> Convert7/1
  Reinterpret3/1 -> ri_to_c5/1
  Reinterpret2/1 -> ri_to_c5/2
  Convert8/1 -> Reinterpret4/1
  Convert10/1 -> Reinterpret6/1
  c_to_ri2/2 -> Convert8/1
  c_to_ri2/1 -> Convert10/1
  Reinterpret6/1 -> ri_to_c6/1
  Reinterpret4/1 -> ri_to_c6/2
  Convert11/1 -> Reinterpret7/1
  Convert12/1 -> Reinterpret8/1
  c_to_ri3/2 -> Convert11/1
  c_to_ri3/1 -> Convert12/1
  Reinterpret8/1 -> ri_to_c7/1
  Reinterpret7/1 -> ri_to_c7/2
  pipeline1/1(q) -> c_to_ri/1
  pipeline2/1(q) -> c_to_ri1/1
  pipeline3/1(q) -> c_to_ri2/1
  pipeline4/1(q) -> c_to_ri3/1
  ri_to_c7/1 -> fft1/6(in03)
  ri_to_c6/1 -> fft1/5(in02)
  ri_to_c5/1 -> fft1/4(in01)
  ri_to_c4/1 -> fft1/3(in00)
  [fftsyncin] -> pfb_fir/1(sync)
  rein_s_b15_0/1 -> Mux13/3
  rein_s_b15_2/1 -> Mux15/3
  rein_s_b15_3/1 -> Mux16/3
  rein_s_b15_4/1 -> Mux17/3
  rein_s_b15_5/1 -> Mux18/3
  rein_s_b15_6/1 -> Mux19/3
  rein_s_b15_7/1 -> Mux20/3
  Mux14/1 -> [daci1]
  Mux15/1 -> [daci2]
  Mux16/1 -> [daci3]
  Mux17/1 -> [dacq0]
  Mux18/1 -> [dacq1]
  Mux20/1 -> [dacq3]
  Mux19/1 -> [dacq2]
  From Workspace11/1 -> testFreq/1(sim_reg)
  [useTestFreq] -> Mux20/1, Mux19/1, Mux18/1, Mux17/1, Mux16/1, Mux15/1, Mux14/1, Mux13/1
  [resetDAC] -> dac_mkid_4x/13
  count_2bit/1 -> stffts_fsm/1(out_reg), mux_en_nextstate/1, Gateway Out25/1, mux_output_fftsync/1
  mux_en_nextstate/1 -> count_2bit/2
  Constant7/1 -> mux_en_nextstate/5
  Constant24/1 -> mux_output_fftsync/4, mux_output_fftsync/3, mux_output_fftsync/2
  Constant25/1 -> Delay21/1, mux_output_fftsync/5
  Constant26/1 -> mux_en_nextstate/3
  DRAM_LUT/9(sync_out) -> [lut_sync]
  [lut_sync] -> Gateway Out26/1, mux_en_nextstate/4
  [startFFTs] -> Gateway Out24/1, Delay19/1, count_2bit/1
  posedge1/1 -> [fftsyncin]
  [run_ffts] -> posedge1/1
  fftshift/1(in_reg) -> bits_0_11_/1
  bits_0_11_/1 -> [fftmask]
  stffts_fsm/1(sim_out) -> Terminator10/1
  mux_output_fftsync/1 -> [run_ffts], Gateway Out27/1
  From Workspace5/1 -> fftsynctime/1(sim_reg)
  fftsynctime/1(in_reg) -> Relational1/1
  BinData/1(data_out) -> fifoassign6_3/1, fifoassign6_2/1, fifoassign6_1/1, fifoassign6_/1, coefbit3_/1, coefbit2_/1, coefbit1_/1, coefbit0_/1
  Logical1/1 -> [fftcoefsync], BinCounter/1
  [fftsyncout] -> Logical1/1
  wr_coef0/1 -> Gateway Out8/1, [fftwesync]
  BinCounter/1 -> [fftbinnumber], bincount_out/1(out_reg), Gateway Out14/1, BinData/1(addr), Relational4/2, Relational1/2
  Constant1/1 -> BinData/2(data_in)
  Constant20/1 -> BinData/3(we)
  Relational1/1 -> [fftlastbin], Logical1/2
  coefbit0_/1 -> wr_coef0/2
  [fftsyncout] -> Register/3
  [run_ffts] -> Inverter8/1, Register/1, Gateway Out15/1
  Register/1 -> Delay/1
  Logical4/1 -> coefWrEn_and_validbin/1, [fftcoefwren]
  Inverter8/1 -> Register/2
  numffts/1(in_reg) -> Relational3/1
  [fftcoefsync] -> Logical5/1
  [fftsyncin] -> fftcounter/1
  fftcounter/1 -> Gateway Out13/1, fftcounter_out/1(out_reg), Relational3/2
  From Workspace4/1 -> numffts/1(sim_reg)
  Delay/1 -> [run_ffts_sync], Logical4/2, Logical6/2
  Logical16/1 -> Logical15/1, Logical5/2, [fftcnt_done]
  fftcounter_out/1(sim_out) -> Terminator2/1
  bincount_out/1(sim_out) -> Terminator9/1
  Logical5/1 -> Logical6/1
  Logical6/1 -> timestamper/2, fftcounter/2
  coefbit1_/1 -> wr_coef1/2
  coefbit2_/1 -> wr_coef2/2
  coefbit3_/1 -> wr_coef3/2
  wr_coef1/1 -> Gateway Out9/1, [fftwesync1]
  wr_coef2/1 -> Gateway Out10/1, [fftwesync2]
  wr_coef3/1 -> Gateway Out11/1, [fftwesync3]
  maxNumBins/1 -> Relational4/1
  Relational4/1 -> coefWrEn_and_validbin/2
  coefWrEn_and_validbin/1 -> wr_coef3/1, wr_coef2/1, wr_coef1/1, wr_coef0/1
  fifoassign6_/1 -> Gateway Out12/1, [fifo_wr_addr]
  [fifo_wr_addr] -> RectToPolar/3(chan)
  [fftwesync] -> RectToPolar/1(dvld_in)
  [fifo_wr_addr1] -> RectToPolar1/3(chan)
  [fftwesync1] -> RectToPolar1/1(dvld_in)
  [mainRst] -> FIFO64_1/6(rst)
  RectToPolar/2(cmplx_dout) -> FIFO64_1/3(din)
  RectToPolar/1(dvld_out) -> FIFO64_1/2(wr)
  RectToPolar/3(chandly) -> FIFO64_1/1(chanwr)
  zero_bool_3/1 -> FIFO64_1/8(wren), FIFO64_1/7(rden)
  zero_bool_1/1 -> FIFO64_/8(wren), FIFO64_/7(rden)
  [mainRst] -> FIFO64_/6(rst)
  RectToPolar1/1(dvld_out) -> FIFO64_/2(wr)
  RectToPolar1/3(chandly) -> FIFO64_/1(chanwr)
  RectToPolar1/2(cmplx_dout) -> FIFO64_/3(din)
  [dumpFifo] -> MCode1/1
  MCode1/1 -> Assert/1
  MCode1/4 -> [chanrd]
  MCode1/2 -> Assert1/1
  MCode1/3 -> [wr_data_sel]
  [chanfifo_empty] -> bool_/1
  [mainRst] -> bool_4/1
  [proc_busy] -> bool_5/1
  [is_pulse] -> bool_6/1
  [pulse_dvld] -> bool_7/1
  [chanfifo_halffull] -> bool_2/1, bool_1/1
  Assert/1 -> [rd]
  Assert1/1 -> [wr_out_data]
  bool_/1 -> MCode1/2
  bool_1/1 -> MCode1/3
  bool_2/1 -> MCode1/4
  bool_4/1 -> MCode1/6
  bool_5/1 -> MCode1/7
  bool_6/1 -> MCode1/8
  bool_7/1 -> MCode1/9
  MCode1/6 -> [state]
  MCode1/7 -> [clear_pulse]
  lastChanToRead/1(in_reg) -> MCode1/10
  MCode1/8 -> [datapath_enable]
  MCode1/9 -> [save_event]
  MCode1/10 -> [delete_event]
  [ram_pulse_out] -> bool_8/1
  MCode1/11 -> [ram_pulse_wr]
  bool_8/1 -> MCode1/12
  lsb0_5_1/1 -> [fifo_rd_addr]
  [chanrd] -> bits76_/1, lsb0_5_1/1
  bits76_/1 -> [fifosel]
  zero_bool_5/1 -> MCode1/5
  From Workspace3/1 -> lastChanToRead/1(sim_reg)
  [is_calc_mean] -> MCode1/13
  [is_write_raw_data] -> MCode1/11
  MCode1/12 -> [calc_mean]
  MCode1/13 -> [store_mean]
  FIFO64_1/1(q) -> datamux/2
  FIFO64_/1(q) -> datamux/3
  FIFO64_1/2(empty) -> emptymux/2
  FIFO64_/2(empty) -> emptymux/3
  FIFO64_1/3(halffull) -> quartfull/2
  FIFO64_/3(halffull) -> quartfull/3
  FIFO64_/8(dvld) -> vldmux/3
  FIFO64_1/8(dvld) -> vldmux/2
  [fifosel] -> Delay18/1
  vldmux/1 -> Delay20/1
  quartfull/1 -> [chanfifo_halffull]
  emptymux/1 -> [chanfifo_empty]
  datamux/1 -> [chanfifo_q]
  Delay18/1 -> emptymux/1, vldmux/1, quartfull/1, datamux/1
  [fifo_rd_addr] -> FIFO64_/4(chanrd)
  [fiford1] -> FIFO64_/5(rd)
  [fiford0] -> FIFO64_1/5(rd)
  [fifo_rd_addr] -> FIFO64_1/4(chanrd)
  bit0/1 -> [mainRst]
  bit4/1 -> [startDac]
  bit1/1 -> [stFFTMem]
  statusFlags/1(sim_out) -> Terminator8/1
  Concat/1 -> statusFlags/1(out_reg)
  Constant10/1 -> Concat/1, Concat/2, Concat/3, Concat/4
  [adcwavememDone] -> Concat/15
  bit7/1 -> [adcwavememStart]
  bit8/1 -> [adcwavememWE]
  bit9__/1 -> [adcwavememSel]
  controlReg/1(in_reg) -> bit1/1, bit26/1, bit25/1, bit24/1, bit23/1, bit22/1, bit21/1, bit20/1, bit19/1, bit18/1, bit17/1, bit16/1, bit15/1, bit14/1, bit13/1, bit12/1, bit9__/1, bit8/1, bit7/1, bit6/1, bit5/1, bit4/1, bit3/1, bit2/1, bit0/1
  [adcvalid] -> Concat/14
  bit12/1 -> [adcforcesync]
  bit13/1 -> [dacLoopBack]
  bit2/1 -> [fftMemWE]
  bit3/1 -> [seeaddress]
  From Workspace/1 -> controlReg/1(sim_reg)
  bit14/1 -> [useTestFreq]
  bit15/1 -> [resetDAC]
  bit16/1 -> [dumpFifo]
  bit6/1 -> [startFFTs]
  [run_ffts] -> Concat/13
  [fftcnt_done] -> Concat/9
  [outMemDone] -> Concat/16
  bit5/1 -> [is_write_raw_data]
  bit17/1 -> [clearPhase]
  [chanfifo_dvld] -> PhaseCorrect1/1(dvld_in)
  PhaseCorrect1/1(dvld_out) -> [phaserot_dvld]
  PhaseCorrect1/2(cmplx_dout) -> [phaserot_data]
  [chanrd] -> PhaseCorrect1/3(chan)
  [datapath_enable] -> PhaseCorrect1/4(en)
  [clearPhase] -> PhaseCorrect1/5(clrPhase)
  [chanfifo_q] -> PhaseCorrect1/2(cmplx_din)
  [phaserot_dvld] -> PulseDetector/1(dvld_in)
  [phaserot_data] -> PulseDetector/2(din)
  PulseDetector/2(dvld_out) -> Assert2/1
  PulseDetector/3(busy) -> Assert3/1
  PulseDetector/4(pulse) -> [is_pulse]
  PulseDetector/5(detect) -> [pulse_detect]
  Assert3/1 -> [proc_busy]
  Assert2/1 -> [pulse_dvld]
  [clear_pulse] -> PulseDetector/3(clear)
  [datapath_enable] -> PulseDetector/4(en)
  [chanrd] -> PulseDetector/5(chan)
  PulseDetector/6(savedpulsestate) -> [ram_pulse_out]
  [ram_pulse_wr] -> PulseDetector/6(savepulsestate)
  PulseDetector/1(datadly) -> [pulse_dout]
  ui32_/1 -> Mux21/2
  Concat2/1 -> Mux21/3
  Concat1/1 -> Mux21/4
  [chanrd] -> lsb8_/1
  Concat4/1 -> Mux21/5
  Mux21/1 -> [chan_fifo_q_mux]
  [wr_data_sel] -> Mux21/1
  lsb8_/1 -> Concat1/4
  OutFIFO/1 -> c2Polar16_2/1(c), TSLow1/1, TSHi1/1, MemRecordPolar/2(DataIn)
  Logical/1 -> OutFIFO/3, Gateway Out20/1, MemRecordPolar/3(WE)
  OutFIFO/2 -> Inverter/1
  MemRecordPolar/1(memDone) -> Gateway Out21/1, [outMemDone]
  [outMemDone] -> Inverter6/1
  Inverter/1 -> [fifo_data_avail], Gateway Out18/1
  [fifo_data_avail] -> Logical/1
  Inverter6/1 -> Logical/3
  [chan_fifo_q_mux] -> SinglaEvtFIFO1/1
  [wr_out_data] -> SinglaEvtFIFO1/2
  SinglaEvtFIFO1/1 -> OutFIFO/1
  EventLength/1 -> EventSaveFSM/3
  zero_bool_6/1 -> EventSaveFSM/4
  EventSaveFSM/1 -> Gateway Out16/1, SinglaEvtFIFO1/3
  [delete_event] -> Logical2/2, Mux23/2, Gateway Out23/1
  [save_event] -> edgdet/1, Logical2/1, Mux22/2, Gateway Out22/1
  EventSaveFSM/2 -> Delay2/1, Gateway Out17/1
  Delay2/1 -> OutFIFO/2
  bit18/1 -> [is_calc_mean]
  From Workspace6/1 -> fftshift/1(sim_reg)
  Gateway Out/1 -> fsmph/1
  Gateway Out1/1 -> fsmph/2
  Gateway Out2/1 -> fsmph/3
  Gateway Out3/1 -> fsmph/4
  Gateway Out4/1 -> fsmph/5
  Gateway Out5/1 -> fsmph/6
  Gateway Out6/1 -> fsmph/7
  Gateway Out7/1 -> fsmph/8
  [state] -> Gateway Out/1
  [dumpFifo] -> Gateway Out1/1
  [flush_input_fifo] -> Gateway Out2/1
  [chanfifo_empty] -> Gateway Out3/1
  [wr_out_data] -> Gateway Out4/1
  [chanrd] -> Gateway Out5/1
  c2polar_/1(power) -> Gateway Out6/1
  c2polar_/2(phase) -> Gateway Out7/1
  [pulse_dout] -> c2polar_/1(c)
  Gateway Out8/1 -> fftscope/1
  Gateway Out9/1 -> fftscope/2
  Gateway Out10/1 -> fftscope/3
  Gateway Out11/1 -> fftscope/4
  Gateway Out12/1 -> fftscope/5
  Gateway Out13/1 -> fftscope/6
  Gateway Out14/1 -> fftscope/7
  Gateway Out15/1 -> fftscope/8
  Gateway Out22/1 -> outmemscope/1
  Gateway Out23/1 -> outmemscope/2
  Gateway Out16/1 -> outmemscope/3
  Gateway Out17/1 -> outmemscope/4
  Gateway Out18/1 -> outmemscope/5
  Gateway Out19/1 -> outmemscope/6
  Gateway Out20/1 -> outmemscope/7
  Gateway Out21/1 -> outmemscope/8
  Gateway Out24/1 -> fsmph1/1
  Gateway Out25/1 -> fsmph1/2
  Gateway Out26/1 -> fsmph1/3
  Gateway Out27/1 -> fsmph1/4
  Gateway Out28/1 -> fsmph1/5
  Gateway Out29/1 -> fsmph1/6
  Gateway Out30/1 -> fsmph1/7
  Gateway Out31/1 -> fsmph1/8
  LUTsize/1(in_reg) -> Gateway Out28/1, [LUTsize]
  [startDac] -> Gateway Out29/1, DRAM_LUT/2(startDAC)
  [mainRst] -> Gateway Out30/1, DRAM_LUT/3(sys_sync)
  DRAM_LUT/1(data_i0) -> Mux13/2, dac_mkid_4x/1
  Delay19/1 -> mux_en_nextstate/2
  Mux13/1 -> Gateway Out31/1, [daci0]
  bit19/1 -> [is_neg_freq]
  Gateway Out38/1 -> outdata1/1
  Gateway Out39/1 -> outdata1/2
  Gateway Out32/1 -> outdata1/3
  Gateway Out33/1 -> outdata1/4
  ui16_1/1 -> Concat2/2
  [is_pulse] -> Concat1/3
  [timestamp_reset] -> timestamper/1
  bit20/1 -> [timestamp_reset]
  timestamper/1 -> timestamp_out/1(out_reg), [timestamp]
  low16_1/1 -> rein_s_b15_1/1
  low16_0/1 -> rein_s_b15_0/1
  low16_2/1 -> rein_s_b15_2/1
  low16_3/1 -> rein_s_b15_3/1
  low16_4/1 -> rein_s_b15_4/1
  low16_5/1 -> rein_s_b15_5/1
  low16_6/1 -> rein_s_b15_6/1
  low16_7/1 -> rein_s_b15_7/1
  rein_s_b15_1/1 -> Mux14/3
  From Workspace12/1 -> testFreq1/1(sim_reg)
  From Workspace13/1 -> testFreq2/1(sim_reg)
  From Workspace14/1 -> testFreq3/1(sim_reg)
  From Workspace15/1 -> testFreq4/1(sim_reg)
  From Workspace16/1 -> testFreq5/1(sim_reg)
  From Workspace17/1 -> testFreq6/1(sim_reg)
  From Workspace18/1 -> testFreq7/1(sim_reg)
  testFreq/1(in_reg) -> low16_0/1
  testFreq1/1(in_reg) -> low16_1/1
  testFreq2/1(in_reg) -> low16_2/1
  testFreq3/1(in_reg) -> low16_3/1
  testFreq4/1(in_reg) -> low16_4/1
  testFreq5/1(in_reg) -> low16_5/1
  testFreq6/1(in_reg) -> low16_6/1
  testFreq7/1(in_reg) -> low16_7/1
  timestamp_out/1(sim_out) -> Terminator1/1
  Gateway Out40/1 -> dacscope/1
  Gateway Out41/1 -> dacscope/2
  Gateway Out42/1 -> dacscope/3
  Gateway Out43/1 -> dacscope/4
  Gateway Out44/1 -> dacscope/5
  Gateway Out45/1 -> dacscope/6
  Gateway Out46/1 -> dacscope/7
  Gateway Out47/1 -> dacscope/8
  [adc_q0] -> Gateway Out41/1
  [adc_i0] -> Gateway Out40/1
  [adc_q1] -> Gateway Out43/1
  [adc_i1] -> Gateway Out42/1
  [adc_q2] -> Gateway Out45/1
  [adc_i2] -> Gateway Out44/1
  [adc_q3] -> Gateway Out47/1
  [adc_i3] -> Gateway Out46/1
  Gateway Out50/1 -> fftscope1/1
  Gateway Out51/1 -> fftscope1/2
  Gateway Out34/1 -> fftscope1/3
  Gateway Out35/1 -> fftscope1/4
  Gateway Out36/1 -> fftscope1/5
  Gateway Out37/1 -> fftscope1/6
  Gateway Out48/1 -> fftscope1/7
  Gateway Out49/1 -> fftscope1/8
  c2polar_3/1(power) -> Gateway Out36/1
  c2polar_3/2(phase) -> Gateway Out37/1
  c2polar_5/1(power) -> Gateway Out48/1
  c2polar_5/2(phase) -> Gateway Out49/1
  c2polar_2/2(phase) -> Gateway Out35/1
  c2polar_2/1(power) -> Gateway Out34/1
  c2polar_1/2(phase) -> Gateway Out51/1
  c2polar_1/1(power) -> Gateway Out50/1
  [fftcoef1] -> RectToPolar1/2(cmplx_din)
  [fftcoef0] -> RectToPolar/2(cmplx_din)
  [fifo_wr_addr2] -> RectToPolar2/3(chan)
  [fftwesync2] -> RectToPolar2/1(dvld_in)
  [fftcoef2] -> RectToPolar2/2(cmplx_din)
  [fifo_wr_addr3] -> RectToPolar3/3(chan)
  [fftwesync3] -> RectToPolar3/1(dvld_in)
  [fftcoef3] -> RectToPolar3/2(cmplx_din)
  [mainRst] -> FIFO64_2/6(rst)
  zero_bool_2/1 -> FIFO64_2/8(wren), FIFO64_2/7(rden)
  [fiford2] -> FIFO64_2/5(rd)
  [fifo_rd_addr] -> FIFO64_2/4(chanrd)
  [mainRst] -> FIFO64_3/6(rst)
  zero_bool_4/1 -> FIFO64_3/8(wren), FIFO64_3/7(rden)
  [fiford3] -> FIFO64_3/5(rd)
  [fifo_rd_addr] -> FIFO64_3/4(chanrd)
  RectToPolar2/3(chandly) -> FIFO64_2/1(chanwr)
  RectToPolar2/1(dvld_out) -> FIFO64_2/2(wr)
  RectToPolar2/2(cmplx_dout) -> FIFO64_2/3(din)
  RectToPolar3/1(dvld_out) -> FIFO64_3/2(wr)
  RectToPolar3/2(cmplx_dout) -> FIFO64_3/3(din)
  RectToPolar3/3(chandly) -> FIFO64_3/1(chanwr)
  bits2_/1 -> Relational/1
  bits2_1/1 -> Relational2/1
  bits2_2/1 -> Relational5/1
  bits2_3/1 -> Relational6/1
  [rd] -> Logical13/2
  [rd] -> Logical12/2
  [rd] -> Logical11/2
  [rd] -> Logical10/2
  Relational/1 -> Logical10/1
  Relational2/1 -> Logical11/1
  Relational5/1 -> Logical12/1
  Relational6/1 -> Logical13/1
  [fifosel] -> Relational6/2
  [fifosel] -> Relational5/2
  [fifosel] -> Relational2/2
  [fifosel] -> Relational/2
  Logical10/1 -> [fiford0]
  Logical11/1 -> [fiford1]
  Logical12/1 -> [fiford2]
  Logical13/1 -> [fiford3]
  FIFO64_2/8(dvld) -> vldmux/4
  FIFO64_3/8(dvld) -> vldmux/5
  FIFO64_2/3(halffull) -> quartfull/4
  FIFO64_3/3(halffull) -> quartfull/5
  FIFO64_2/2(empty) -> emptymux/4
  FIFO64_3/2(empty) -> emptymux/5
  FIFO64_2/1(q) -> datamux/4
  FIFO64_3/1(q) -> datamux/5
  fifoassign6_3/1 -> [fifo_wr_addr3]
  fifoassign6_2/1 -> [fifo_wr_addr2]
  fifoassign6_1/1 -> [fifo_wr_addr1]
  Delay20/1 -> [chanfifo_dvld]
  OutFIFO/3 -> [fifo_data_full]
  [fifo_data_avail] -> Concat/11
  [fifo_data_full] -> Concat/12
  [is_pulse] -> Concat/10
  Mux22/1 -> EventSaveFSM/1
  Mux23/1 -> EventSaveFSM/2
  [drop_all_events] -> Mux23/1, Mux22/1
  bool_100/1 -> Mux22/3
  Logical2/1 -> Mux23/3
  bit21/1 -> [drop_all_events]
  readoutStat/1(sim_out) -> Terminator11/1
  Concat3/1 -> readoutStat/1(out_reg)
  Constant2/1 -> Concat3/6, Concat3/5, Concat3/4, Concat3/3, Concat3/2, Concat3/1
  Constant3/1 -> readoutControl/1(sim_reg)
  bit22/1 -> [bitToDataServer0]
  bit23/1 -> [bitToDataServer1]
  [stFFTMem] -> Concat3/16
  [outMemDone] -> Concat3/15
  [fftMemWE] -> Concat3/14
  [fifo_data_avail] -> Concat3/13
  [bitToDataServer0] -> Concat3/12
  [bitToDataServer1] -> Concat3/11
  [fifo_data_full] -> Concat3/10
  Logical3/1 -> Logical/2
  [fftMemWE] -> Logical3/1
  [stFFTMem] -> Logical14/1
  [stFFTMemDS] -> Logical14/2
  [fftMemWEDS] -> Logical3/2
  readoutControl/1(in_reg) -> DSbit6/1, DSbit5/1, DSbit4/1, DSbit3/1, DSbit2/1, DSbit1/1, DSbit0/1
  DSbit0/1 -> [fftMemWEDS]
  DSbit1/1 -> [stFFTMemDS]
  [fftcnt_done] -> Concat3/7
  [is_pulse] -> Concat3/8
  [run_ffts] -> Concat3/9
  DSbit2/1 -> [bitFromDS0]
  DSbit3/1 -> [bitFromDS1]
  DSbit4/1 -> [bitFromDS2]
  DSbit5/1 -> [bitFromDS3]
  [bitFromDS3] -> Concat/8
  [bitFromDS2] -> Concat/7
  [bitFromDS1] -> Concat/6
  [bitFromDS0] -> Concat/5
  [timestamp] -> TSLow/1, TSHi/1
  [pulse_dout] -> c2TruncatePolar16_1/1(c)
  ui16_10/1 -> Concat4/1
  ui16_2/1 -> Concat4/2
  c2TruncatePolar16_1/1(power) -> ui16_10/1
  c2TruncatePolar16_1/2(phase) -> ui16_2/1
  TSHi/1 -> Concat2/1
  TSLow/1 -> Concat1/2
  restofbits_/1 -> Concat1/1
  TSHi1/1 -> Gateway Out38/1
  TSLow1/1 -> Gateway Out39/1
  c2Polar16_2/1(power) -> Gateway Out32/1
  c2Polar16_2/2(phase) -> Gateway Out33/1
  fifoOverFlowCnt/1(sim_out) -> Terminator12/1
  [fifo_data_full] -> posedge3/1
  posedge3/1 -> overflowcounter/2
  overflowcounter/1 -> fifoOverFlowCnt/1(out_reg)
  DSbit6/1 -> [resetOvCnt]
  [resetOvCnt] -> overflowcounter/1
  Logical14/1 -> Gateway Out19/1, MemRecordPolar/1(Start)
  edgdet/1 -> EvtCnt/2
  bit24/1 -> [resetEvtCounter]
  [resetEvtCounter] -> EvtCnt/1
  EvtCnt/1 -> savedEventCounter/1(out_reg)
  Logical15/1 -> Logical4/1
  [fftrunforever] -> Logical15/2
  bit25/1 -> [fftrunforever]
  Relational3/1 -> Logical16/2
  [fftrunforever] -> Logical16/1
  bit26/1 -> [flush_input_fifo]
  [flush_input_fifo] -> MCode1/14
